simulink model "test_old_est"  (Simulink 6.2)
settings: Solver=ode45  StartTime=0.0  StopTime=10.0  RelTol=1e-3
libraries: xbsIndex_r3 x10, fft_library x1
settings Model: LastModifiedBy=mdexter
settings DebuggingCC: SolverPrmCheckMsg=warning

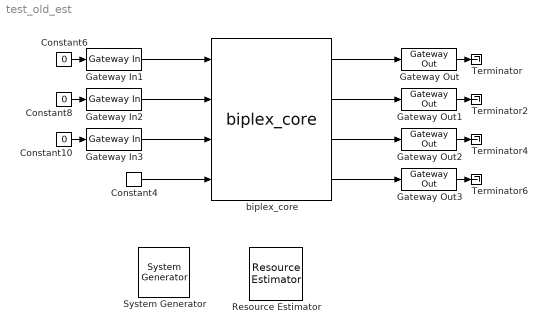
== system test_old_est ==
  " System Generator" : xbsIndex_r3/ System Generator  Tag=genX  xilinxfamily=Virtex2P  part=xc2vp40  speed=-6  package=ff1152  synthesis_tool=XST  directory=./test_old_est.netlist  testbench=off  simulink_period=1  sysclk_period=10  incr_netlist=off  trim_vbits=Everywhere in SubSystem  dbl_ovrd=According to Block Masks  core_generation=According to Block Masks  run_coregen=off  deprecated_control=off  eval_field=0
      settings: AttributesFormatString=System\nGenerator
  Constant10 : Constant  Value=0
  Constant4 : xbsIndex_r3/Constant  const=0  equ=P=C  arith_type=Unsigned  n_bits=10  bin_pt=0  opselect=C  inp2=PCIN>>17  opr=+  inp1=P  carry=CIN  iostate=0  explicit_period=on  period=1  dbl_ovrd=off
  Constant6 : Constant  Value=0
  Constant8 : Constant  Value=0
  Gateway In1 : xbsIndex_r3/Gateway In  arith_type=Unsigned  n_bits=36  bin_pt=0  quantization=Truncate  overflow=Wrap  period=1  timing_constraint=None  locs_specified=off  LOCs={}  needs_fixed_name=off  dbl_ovrd=off  show_param=off
      settings: xl_area=[0 0 0 0 36 0 0]
  Gateway In2 : xbsIndex_r3/Gateway In  arith_type=Unsigned  n_bits=36  bin_pt=0  quantization=Truncate  overflow=Wrap  period=1  timing_constraint=None  locs_specified=off  LOCs={}  needs_fixed_name=off  dbl_ovrd=off  show_param=off
      settings: xl_area=[0 0 0 0 36 0 0]
  Gateway In3 : xbsIndex_r3/Gateway In  arith_type=Boolean  n_bits=8  bin_pt=7  quantization=Truncate  overflow=Wrap  period=1  timing_constraint=None  locs_specified=off  LOCs={}  needs_fixed_name=off  dbl_ovrd=off  show_param=off
      settings: xl_area=[0 0 0 0 1 0 0]
  Gateway Out{,1..3} (4 alike) : xbsIndex_r3/Gateway Out  output_type=Double  nbits=8  bin_pt=6  arith_type=Boolean  quantization=Truncate  overflow=Wrap  hdl_port=on  timing_constraint=None  locs_specified=off  LOCs={}  needs_fixed_name=off  show_param=off
      Gateway Out settings: xl_area=[0 0 0 0 36 0 0]
      Gateway Out1 settings: xl_area=[0 0 0 0 36 0 0]
      Gateway Out2 settings: xl_area=[0 0 0 0 1 0 0]
      Gateway Out3 settings: xl_area=[0 0 0 0 1 0 0]
  Resource Estimator : xbsIndex_r3/Resource Estimator  Tag=resEstTag  xl_estimator_area=[5709 8870 8 9342 147 24 0]  xl_use_estimator_area=off  simulink_period=1  mrp_directory=./test_old_est.netlist
      settings: AttributesFormatString=Resource Estimator\n%<xl_estimator_area>\n[SL FF BR LUT IO MUL TBUF]
  Terminator{,2,4,6} (4 alike) : Terminator
  biplex_core : fft_library/biplex_core  FFTSize=10  BitWidth=18  quantization="Round  (unbiased: +/- Inf)"  overflow=Saturate  add_latency=1  mult_latency=3  bram_latency=1
      link override fft_stage_1/butterfly/Convert: quantization="Round  (unbiased: +/- Inf)"  overflow=Saturate
      link override fft_stage_1/butterfly/Convert1: quantization="Round  (unbiased: +/- Inf)"  overflow=Saturate
      link override fft_stage_1/butterfly/Convert2: quantization="Round  (unbiased: +/- Inf)"  overflow=Saturate
      link override fft_stage_1/butterfly/Convert3: quantization="Round  (unbiased: +/- Inf)"  overflow=Saturate
      link override fft_stage_1/delay_b/delay_bram/Constant2: equ=P=C
      link override fft_stage_1/delay_b/delay_im/delay_bram/Constant2: equ=P=C
      link override fft_stage_1/delay_b/delay_re/delay_bram/Constant2: equ=P=C
      link override fft_stage_1/delay_f/delay_bram/Constant2: equ=P=C
      link override fft_stage_1/delay_f/delay_im/delay_bram/Constant2: equ=P=C
      link override fft_stage_1/delay_f/delay_re/delay_bram/Constant2: equ=P=C
      link override fft_stage_1/sync_delay_x/Constant: equ=P=C
      link override fft_stage_1/sync_delay_x/Constant1: equ=P=C
      link override fft_stage_1/sync_delay_x/Constant2: equ=P=C
      link override fft_stage_1/sync_delay_x/Constant3: equ=P=C
      link override fft_stage_10/butterfly/Convert: quantization="Round  (unbiased: +/- Inf)"  overflow=Saturate
      link override fft_stage_10/butterfly/Convert1: quantization="Round  (unbiased: +/- Inf)"  overflow=Saturate
      link override fft_stage_10/butterfly/Convert2: quantization="Round  (unbiased: +/- Inf)"  overflow=Saturate
      link override fft_stage_10/butterfly/Convert3: quantization="Round  (unbiased: +/- Inf)"  overflow=Saturate
      link override fft_stage_10/butterfly/twiddle_general/br_coeff_gen/ROM: distributed_mem=off
      link override fft_stage_10/butterfly/twiddle_general/br_coeff_gen/ROM1: distributed_mem=off
      link override fft_stage_10/butterfly/twiddle_general_3mult/br_coeff_gen/ROM: distributed_mem=off
      link override fft_stage_10/butterfly/twiddle_general_3mult/br_coeff_gen/ROM1: distributed_mem=off
      link override fft_stage_10/sync_delay_x/Constant: equ=P=C
      link override fft_stage_10/sync_delay_x/Constant1: equ=P=C
      link override fft_stage_10/sync_delay_x/Constant2: equ=P=C
      link override fft_stage_10/sync_delay_x/Constant3: equ=P=C
      link override fft_stage_2/butterfly/Convert: quantization="Round  (unbiased: +/- Inf)"  overflow=Saturate
      link override fft_stage_2/butterfly/Convert1: quantization="Round  (unbiased: +/- Inf)"  overflow=Saturate
      link override fft_stage_2/butterfly/Convert2: quantization="Round  (unbiased: +/- Inf)"  overflow=Saturate
      link override fft_stage_2/butterfly/Convert3: quantization="Round  (unbiased: +/- Inf)"  overflow=Saturate
      link override fft_stage_2/delay_b/delay_bram/Constant2: equ=P=C
      link override fft_stage_2/delay_b/delay_im/delay_bram/Constant2: equ=P=C
      link override fft_stage_2/delay_b/delay_re/delay_bram/Constant2: equ=P=C
      link override fft_stage_2/delay_f/delay_bram/Constant2: equ=P=C
      link override fft_stage_2/delay_f/delay_im/delay_bram/Constant2: equ=P=C
      link override fft_stage_2/delay_f/delay_re/delay_bram/Constant2: equ=P=C
      link override fft_stage_2/sync_delay_x/Constant: equ=P=C
      link override fft_stage_2/sync_delay_x/Constant1: equ=P=C
      link override fft_stage_2/sync_delay_x/Constant2: equ=P=C
      link override fft_stage_2/sync_delay_x/Constant3: equ=P=C
      link override fft_stage_3/butterfly/Convert: quantization="Round  (unbiased: +/- Inf)"  overflow=Saturate
      link override fft_stage_3/butterfly/Convert1: quantization="Round  (unbiased: +/- Inf)"  overflow=Saturate
      link override fft_stage_3/butterfly/Convert2: quantization="Round  (unbiased: +/- Inf)"  overflow=Saturate
      link override fft_stage_3/butterfly/Convert3: quantization="Round  (unbiased: +/- Inf)"  overflow=Saturate
      link override fft_stage_3/delay_b/delay_im/delay_bram/Constant2: equ=P=C
      link override fft_stage_3/delay_b/delay_re/delay_bram/Constant2: equ=P=C
      link override fft_stage_3/delay_f/delay_im/delay_bram/Constant2: equ=P=C
      link override fft_stage_3/delay_f/delay_re/delay_bram/Constant2: equ=P=C
      link override fft_stage_3/sync_delay_x/Constant: equ=P=C
      link override fft_stage_3/sync_delay_x/Constant1: equ=P=C
      link override fft_stage_3/sync_delay_x/Constant2: equ=P=C
      link override fft_stage_3/sync_delay_x/Constant3: equ=P=C
      link override fft_stage_4/butterfly/Convert: quantization="Round  (unbiased: +/- Inf)"  overflow=Saturate
      link override fft_stage_4/butterfly/Convert1: quantization="Round  (unbiased: +/- Inf)"  overflow=Saturate
      link override fft_stage_4/butterfly/Convert2: quantization="Round  (unbiased: +/- Inf)"  overflow=Saturate
      link override fft_stage_4/butterfly/Convert3: quantization="Round  (unbiased: +/- Inf)"  overflow=Saturate
      link override fft_stage_4/delay_b/delay_im/delay_bram/Constant2: equ=P=C
      link override fft_stage_4/delay_b/delay_re/delay_bram/Constant2: equ=P=C
      link override fft_stage_4/delay_f/delay_im/delay_bram/Constant2: equ=P=C
      link override fft_stage_4/delay_f/delay_re/delay_bram/Constant2: equ=P=C
      link override fft_stage_4/sync_delay_x/Constant: equ=P=C
      link override fft_stage_4/sync_delay_x/Constant1: equ=P=C
      link override fft_stage_4/sync_delay_x/Constant2: equ=P=C
      link override fft_stage_4/sync_delay_x/Constant3: equ=P=C
      link override fft_stage_5/butterfly/Convert: quantization="Round  (unbiased: +/- Inf)"  overflow=Saturate
      link override fft_stage_5/butterfly/Convert1: quantization="Round  (unbiased: +/- Inf)"  overflow=Saturate
      link override fft_stage_5/butterfly/Convert2: quantization="Round  (unbiased: +/- Inf)"  overflow=Saturate
      link override fft_stage_5/butterfly/Convert3: quantization="Round  (unbiased: +/- Inf)"  overflow=Saturate
      link override fft_stage_5/sync_delay_x/Constant: equ=P=C
      link override fft_stage_5/sync_delay_x/Constant1: equ=P=C
      link override fft_stage_5/sync_delay_x/Constant2: equ=P=C
      link override fft_stage_5/sync_delay_x/Constant3: equ=P=C
      link override fft_stage_6/butterfly/Convert: quantization="Round  (unbiased: +/- Inf)"  overflow=Saturate
      link override fft_stage_6/butterfly/Convert1: quantization="Round  (unbiased: +/- Inf)"  overflow=Saturate
      link override fft_stage_6/butterfly/Convert2: quantization="Round  (unbiased: +/- Inf)"  overflow=Saturate
      link override fft_stage_6/butterfly/Convert3: quantization="Round  (unbiased: +/- Inf)"  overflow=Saturate
      link override fft_stage_6/sync_delay_x/Constant: equ=P=C
      link override fft_stage_6/sync_delay_x/Constant1: equ=P=C
      link override fft_stage_6/sync_delay_x/Constant2: equ=P=C
      link override fft_stage_6/sync_delay_x/Constant3: equ=P=C
      link override fft_stage_7/butterfly/Convert: quantization="Round  (unbiased: +/- Inf)"  overflow=Saturate
      link override fft_stage_7/butterfly/Convert1: quantization="Round  (unbiased: +/- Inf)"  overflow=Saturate
      link override fft_stage_7/butterfly/Convert2: quantization="Round  (unbiased: +/- Inf)"  overflow=Saturate
      link override fft_stage_7/butterfly/Convert3: quantization="Round  (unbiased: +/- Inf)"  overflow=Saturate
      link override fft_stage_7/sync_delay_x/Constant: equ=P=C
      link override fft_stage_7/sync_delay_x/Constant1: equ=P=C
      link override fft_stage_7/sync_delay_x/Constant2: equ=P=C
      link override fft_stage_7/sync_delay_x/Constant3: equ=P=C
      link override fft_stage_8/butterfly/Convert: quantization="Round  (unbiased: +/- Inf)"  overflow=Saturate
      link override fft_stage_8/butterfly/Convert1: quantization="Round  (unbiased: +/- Inf)"  overflow=Saturate
      link override fft_stage_8/butterfly/Convert2: quantization="Round  (unbiased: +/- Inf)"  overflow=Saturate
      link override fft_stage_8/butterfly/Convert3: quantization="Round  (unbiased: +/- Inf)"  overflow=Saturate
      link override fft_stage_8/sync_delay_x/Constant: equ=P=C
      link override fft_stage_8/sync_delay_x/Constant1: equ=P=C
      link override fft_stage_8/sync_delay_x/Constant2: equ=P=C
      link override fft_stage_8/sync_delay_x/Constant3: equ=P=C
      link override fft_stage_9/butterfly/Convert: quantization="Round  (unbiased: +/- Inf)"  overflow=Saturate
      link override fft_stage_9/butterfly/Convert1: quantization="Round  (unbiased: +/- Inf)"  overflow=Saturate
      link override fft_stage_9/butterfly/Convert2: quantization="Round  (unbiased: +/- Inf)"  overflow=Saturate
      link override fft_stage_9/butterfly/Convert3: quantization="Round  (unbiased: +/- Inf)"  overflow=Saturate
      link override fft_stage_9/butterfly/twiddle_general/br_coeff_gen/ROM: distributed_mem=off
      link override fft_stage_9/butterfly/twiddle_general/br_coeff_gen/ROM1: distributed_mem=off
      link override fft_stage_9/butterfly/twiddle_general_3mult/br_coeff_gen/ROM: distributed_mem=off
      link override fft_stage_9/butterfly/twiddle_general_3mult/br_coeff_gen/ROM1: distributed_mem=off
      link override fft_stage_9/sync_delay_x/Constant: equ=P=C
      link override fft_stage_9/sync_delay_x/Constant1: equ=P=C
      link override fft_stage_9/sync_delay_x/Constant2: equ=P=C
      link override fft_stage_9/sync_delay_x/Constant3: equ=P=C
      link override fft_stage_1/Counter: xl_area=[5 10 0 10 0 0 0]
      link override fft_stage_1/Delay: xl_area=[1 1 0 0 0 0 0]
      link override fft_stage_1/Mux: xl_area=[18 36 0 36 0 0 0]
      link override fft_stage_1/Mux1: xl_area=[18 36 0 36 0 0 0]
      link override fft_stage_1/butterfly/AddSub: xl_area=[10 19 0 19 0 0 0]
      link override fft_stage_1/butterfly/AddSub1: xl_area=[10 19 0 19 0 0 0]
      link override fft_stage_1/butterfly/AddSub2: xl_area=[10 19 0 19 0 0 0]
      link override fft_stage_1/butterfly/AddSub3: xl_area=[10 19 0 19 0 0 0]
      link override fft_stage_1/butterfly/Convert: xl_area=[29 18 0 57 0 0 0]
      link override fft_stage_1/butterfly/Convert1: xl_area=[29 18 0 57 0 0 0]
      link override fft_stage_1/butterfly/Convert2: xl_area=[29 18 0 57 0 0 0]
      link override fft_stage_1/butterfly/Convert3: xl_area=[29 18 0 57 0 0 0]
      link override fft_stage_1/butterfly/Delay: xl_area=[1 1 0 1 0 0 0]
      link override fft_stage_1/butterfly/Delay3: xl_area=[1 1 0 0 0 0 0]
      link override fft_stage_1/butterfly/Inverter: xl_area=[0 0 0 0 0 0 0]
      link override fft_stage_1/butterfly/Logical: xl_area=[1 1 0 1 0 0 0]
      link override fft_stage_1/butterfly/Logical1: xl_area=[1 1 0 1 0 0 0]
      link override fft_stage_1/butterfly/Logical10: xl_area=[1 1 0 1 0 0 0]
      link override fft_stage_1/butterfly/Logical11: xl_area=[1 1 0 1 0 0 0]
      link override fft_stage_1/butterfly/Logical12: xl_area=[1 1 0 1 0 0 0]
      link override fft_stage_1/butterfly/Logical13: xl_area=[1 1 0 1 0 0 0]
      link override fft_stage_1/butterfly/Logical2: xl_area=[1 1 0 1 0 0 0]
      link override fft_stage_1/butterfly/Logical3: xl_area=[1 1 0 1 0 0 0]
      link override fft_stage_1/butterfly/Logical4: xl_area=[1 1 0 1 0 0 0]
      link override fft_stage_1/butterfly/Logical5: xl_area=[1 1 0 1 0 0 0]
      link override fft_stage_1/butterfly/Logical6: xl_area=[1 1 0 1 0 0 0]
      link override fft_stage_1/butterfly/Logical7: xl_area=[1 1 0 1 0 0 0]
      link override fft_stage_1/butterfly/Logical8: xl_area=[1 1 0 1 0 0 0]
      link override fft_stage_1/butterfly/Logical9: xl_area=[1 1 0 1 0 0 0]
      link override fft_stage_1/butterfly/Mux: xl_area=[10 20 0 20 0 0 0]
      link override fft_stage_1/butterfly/Mux1: xl_area=[10 20 0 20 0 0 0]
      link override fft_stage_1/butterfly/Mux2: xl_area=[10 20 0 20 0 0 0]
      link override fft_stage_1/butterfly/Mux3: xl_area=[10 20 0 20 0 0 0]
      link override fft_stage_1/delay_b/delay_bram/Counter: xl_area=[7 9 0 12 0 0 0]
      link override fft_stage_1/delay_b/delay_bram/Single Port RAM: xl_area=[0 0 1 0 0 0 0]
      link override fft_stage_1/delay_b/delay_im/delay_bram/Counter: xl_area=[7 9 0 12 0 0 0]
      link override fft_stage_1/delay_b/delay_im/delay_bram/Single Port RAM: xl_area=[0 0 1 0 0 0 0]
      link override fft_stage_1/delay_b/delay_re/delay_bram/Counter: xl_area=[7 9 0 12 0 0 0]
      link override fft_stage_1/delay_b/delay_re/delay_bram/Single Port RAM: xl_area=[0 0 1 0 0 0 0]
      link override fft_stage_1/delay_f/delay_bram/Counter: xl_area=[7 9 0 12 0 0 0]
      link override fft_stage_1/delay_f/delay_bram/Single Port RAM: xl_area=[0 0 1 0 0 0 0]
      link override fft_stage_1/delay_f/delay_im/delay_bram/Counter: xl_area=[7 9 0 12 0 0 0]
      link override fft_stage_1/delay_f/delay_im/delay_bram/Single Port RAM: xl_area=[0 0 1 0 0 0 0]
      link override fft_stage_1/delay_f/delay_re/delay_bram/Counter: xl_area=[7 9 0 12 0 0 0]
      link override fft_stage_1/delay_f/delay_re/delay_bram/Single Port RAM: xl_area=[0 0 1 0 0 0 0]
      link override fft_stage_1/sync_delay_x/Counter: xl_area=[6 10 0 11 0 0 0]
      link override fft_stage_1/sync_delay_x/Logical: xl_area=[1 0 0 1 0 0 0]
      link override fft_stage_1/sync_delay_x/Mux: xl_area=[1 0 0 1 0 0 0]
      link override fft_stage_1/sync_delay_x/Relational: xl_area=[3 0 0 5 0 0 0]
      link override fft_stage_1/sync_delay_x/Relational1: xl_area=[3 0 0 5 0 0 0]
      link override fft_stage_10/Counter: xl_area=[2 1 0 1 0 0 0]
      link override fft_stage_10/Delay: xl_area=[1 1 0 0 0 0 0]
      link override fft_stage_10/Logical1: xl_area=[1 1 0 1 0 0 0]
      link override fft_stage_10/Mux: xl_area=[18 36 0 36 0 0 0]
      link override fft_stage_10/Mux1: xl_area=[18 36 0 36 0 0 0]
      link override fft_stage_10/butterfly/AddSub: xl_area=[12 23 0 23 0 0 0]
      link override fft_stage_10/butterfly/AddSub1: xl_area=[12 23 0 23 0 0 0]
      link override fft_stage_10/butterfly/AddSub2: xl_area=[12 23 0 23 0 0 0]
      link override fft_stage_10/butterfly/AddSub3: xl_area=[12 23 0 23 0 0 0]
      link override fft_stage_10/butterfly/Convert: xl_area=[31 18 0 61 0 0 0]
      link override fft_stage_10/butterfly/Convert1: xl_area=[31 18 0 61 0 0 0]
      link override fft_stage_10/butterfly/Convert2: xl_area=[31 18 0 61 0 0 0]
      link override fft_stage_10/butterfly/Convert3: xl_area=[31 18 0 61 0 0 0]
      link override fft_stage_10/butterfly/Delay: xl_area=[1 1 0 1 0 0 0]
      link override fft_stage_10/butterfly/Delay3: xl_area=[1 1 0 0 0 0 0]
      link override fft_stage_10/butterfly/Inverter: xl_area=[0 0 0 0 0 0 0]
      link override fft_stage_10/butterfly/Logical: xl_area=[1 1 0 1 0 0 0]
      link override fft_stage_10/butterfly/Logical1: xl_area=[1 1 0 1 0 0 0]
      link override fft_stage_10/butterfly/Logical10: xl_area=[1 1 0 1 0 0 0]
      link override fft_stage_10/butterfly/Logical11: xl_area=[1 1 0 1 0 0 0]
      link override fft_stage_10/butterfly/Logical12: xl_area=[1 1 0 1 0 0 0]
      link override fft_stage_10/butterfly/Logical13: xl_area=[1 1 0 1 0 0 0]
      link override fft_stage_10/butterfly/Logical2: xl_area=[1 1 0 1 0 0 0]
      link override fft_stage_10/butterfly/Logical3: xl_area=[1 1 0 1 0 0 0]
      link override fft_stage_10/butterfly/Logical4: xl_area=[1 1 0 1 0 0 0]
      link override fft_stage_10/butterfly/Logical5: xl_area=[1 1 0 1 0 0 0]
      link override fft_stage_10/butterfly/Logical6: xl_area=[1 1 0 1 0 0 0]
      link override fft_stage_10/butterfly/Logical7: xl_area=[1 1 0 1 0 0 0]
      link override fft_stage_10/butterfly/Logical8: xl_area=[1 1 0 1 0 0 0]
      link override fft_stage_10/butterfly/Logical9: xl_area=[1 1 0 1 0 0 0]
      link override fft_stage_10/butterfly/Mux: xl_area=[12 24 0 24 0 0 0]
      link override fft_stage_10/butterfly/Mux1: xl_area=[12 24 0 24 0 0 0]
      link override fft_stage_10/butterfly/Mux2: xl_area=[12 24 0 24 0 0 0]
      link override fft_stage_10/butterfly/Mux3: xl_area=[12 24 0 24 0 0 0]
      link override fft_stage_10/butterfly/twiddle_general/AddSub: xl_area=[11 21 0 21 0 0 0]
      link override fft_stage_10/butterfly/twiddle_general/AddSub1: xl_area=[11 21 0 21 0 0 0]
      link override fft_stage_10/butterfly/twiddle_general/Convert: xl_area=[0 0 0 0 0 0 0]
      link override fft_stage_10/butterfly/twiddle_general/Convert1: xl_area=[0 0 0 0 0 0 0]
      link override fft_stage_10/butterfly/twiddle_general/Convert2: xl_area=[0 0 0 0 0 0 0]
      link override fft_stage_10/butterfly/twiddle_general/Convert3: xl_area=[0 0 0 0 0 0 0]
      link override fft_stage_10/butterfly/twiddle_general/Delay: xl_area=[18 36 0 36 0 0 0]
      link override fft_stage_10/butterfly/twiddle_general/Delay1: xl_area=[18 36 0 0 0 0 0]
      link override fft_stage_10/butterfly/twiddle_general/Delay2: xl_area=[1 1 0 1 0 0 0]
      link override fft_stage_10/butterfly/twiddle_general/Mult: xl_area=[36 72 0 36 0 1 0]
      link override fft_stage_10/butterfly/twiddle_general/Mult1: xl_area=[36 72 0 36 0 1 0]
      link override fft_stage_10/butterfly/twiddle_general/Mult2: xl_area=[36 72 0 36 0 1 0]
      link override fft_stage_10/butterfly/twiddle_general/Mult3: xl_area=[36 72 0 36 0 1 0]
      link override fft_stage_10/butterfly/twiddle_general/br_coeff_gen/Counter: xl_area=[5 9 0 9 0 0 0]
      link override fft_stage_10/butterfly/twiddle_general/br_coeff_gen/ROM: xl_area=[0 0 1 0 0 0 0]
      link override fft_stage_10/butterfly/twiddle_general/br_coeff_gen/ROM1: xl_area=[0 0 1 0 0 0 0]
      link override fft_stage_10/butterfly/twiddle_general_3mult/AddSub: xl_area=[11 22 0 22 0 0 0]
      link override fft_stage_10/butterfly/twiddle_general_3mult/AddSub1: xl_area=[10 19 0 19 0 0 0]
      link override fft_stage_10/butterfly/twiddle_general_3mult/AddSub2: xl_area=[10 19 0 19 0 0 0]
      link override fft_stage_10/butterfly/twiddle_general_3mult/AddSub3: xl_area=[10 19 0 19 0 0 0]
      link override fft_stage_10/butterfly/twiddle_general_3mult/AddSub4: xl_area=[11 22 0 22 0 0 0]
      link override fft_stage_10/butterfly/twiddle_general_3mult/Convert: xl_area=[0 0 0 0 0 0 0]
      link override fft_stage_10/butterfly/twiddle_general_3mult/Convert1: xl_area=[0 0 0 0 0 0 0]
      link override fft_stage_10/butterfly/twiddle_general_3mult/Convert2: xl_area=[0 0 0 0 0 0 0]
      link override fft_stage_10/butterfly/twiddle_general_3mult/Convert3: xl_area=[0 0 0 0 0 0 0]
      link override fft_stage_10/butterfly/twiddle_general_3mult/Convert4: xl_area=[0 0 0 0 0 0 0]
      link override fft_stage_10/butterfly/twiddle_general_3mult/Convert5: xl_area=[0 0 0 0 0 0 0]
      link override fft_stage_10/butterfly/twiddle_general_3mult/Delay: xl_area=[18 36 0 36 0 0 0]
      link override fft_stage_10/butterfly/twiddle_general_3mult/Delay1: xl_area=[18 36 0 0 0 0 0]
      link override fft_stage_10/butterfly/twiddle_general_3mult/Delay2: xl_area=[1 1 0 1 0 0 0]
      link override fft_stage_10/butterfly/twiddle_general_3mult/Delay3: xl_area=[9 18 0 0 0 0 0]
      link override fft_stage_10/butterfly/twiddle_general_3mult/Delay4: xl_area=[9 18 0 0 0 0 0]
      link override fft_stage_10/butterfly/twiddle_general_3mult/Delay5: xl_area=[9 18 0 0 0 0 0]
      link override fft_stage_10/butterfly/twiddle_general_3mult/Mult: xl_area=[36 72 0 36 0 1 0]
      link override fft_stage_10/butterfly/twiddle_general_3mult/Mult1: xl_area=[36 72 0 36 0 1 0]
      link override fft_stage_10/butterfly/twiddle_general_3mult/Mult2: xl_area=[36 72 0 36 0 1 0]
      link override fft_stage_10/butterfly/twiddle_general_3mult/br_coeff_gen/Counter: xl_area=[5 9 0 9 0 0 0]
      link override fft_stage_10/butterfly/twiddle_general_3mult/br_coeff_gen/ROM: xl_area=[0 0 1 0 0 0 0]
      link override fft_stage_10/butterfly/twiddle_general_3mult/br_coeff_gen/ROM1: xl_area=[0 0 1 0 0 0 0]
      link override fft_stage_10/delay_b/delay_im/delay_slr/delay_slr: xl_area=[9 18 0 0 0 0 0]
      link override fft_stage_10/delay_b/delay_re/delay_slr/delay_slr: xl_area=[9 18 0 0 0 0 0]
      link override fft_stage_10/delay_b/delay_slr/delay_slr: xl_area=[18 36 0 0 0 0 0]
      link override fft_stage_10/delay_f/delay_im/delay_slr/delay_slr: xl_area=[9 18 0 0 0 0 0]
      link override fft_stage_10/delay_f/delay_re/delay_slr/delay_slr: xl_area=[9 18 0 0 0 0 0]
      link override fft_stage_10/delay_f/delay_slr/delay_slr: xl_area=[18 36 0 0 0 0 0]
      link override fft_stage_10/sync_delay_x/Counter: xl_area=[2 2 0 3 0 0 0]
      link override fft_stage_10/sync_delay_x/Logical: xl_area=[1 0 0 1 0 0 0]
      link override fft_stage_10/sync_delay_x/Mux: xl_area=[1 0 0 1 0 0 0]
      link override fft_stage_10/sync_delay_x/Relational: xl_area=[1 0 0 1 0 0 0]
      link override fft_stage_10/sync_delay_x/Relational1: xl_area=[1 0 0 1 0 0 0]
      link override fft_stage_2/Counter: xl_area=[5 9 0 9 0 0 0]
      link override fft_stage_2/Delay: xl_area=[1 1 0 0 0 0 0]
      link override fft_stage_2/Logical1: xl_area=[1 1 0 1 0 0 0]
      link override fft_stage_2/Mux: xl_area=[18 36 0 36 0 0 0]
      link override fft_stage_2/Mux1: xl_area=[18 36 0 36 0 0 0]
      link override fft_stage_2/butterfly/AddSub: xl_area=[10 19 0 19 0 0 0]
      link override fft_stage_2/butterfly/AddSub1: xl_area=[10 19 0 19 0 0 0]
      link override fft_stage_2/butterfly/AddSub2: xl_area=[10 19 0 19 0 0 0]
      link override fft_stage_2/butterfly/AddSub3: xl_area=[10 19 0 19 0 0 0]
      link override fft_stage_2/butterfly/Convert: xl_area=[29 18 0 57 0 0 0]
      link override fft_stage_2/butterfly/Convert1: xl_area=[29 18 0 57 0 0 0]
      link override fft_stage_2/butterfly/Convert2: xl_area=[29 18 0 57 0 0 0]
      link override fft_stage_2/butterfly/Convert3: xl_area=[29 18 0 57 0 0 0]
      link override fft_stage_2/butterfly/Delay: xl_area=[1 1 0 1 0 0 0]
      link override fft_stage_2/butterfly/Delay3: xl_area=[1 1 0 0 0 0 0]
      link override fft_stage_2/butterfly/Inverter: xl_area=[0 0 0 0 0 0 0]
      link override fft_stage_2/butterfly/Logical: xl_area=[1 1 0 1 0 0 0]
      link override fft_stage_2/butterfly/Logical1: xl_area=[1 1 0 1 0 0 0]
      link override fft_stage_2/butterfly/Logical10: xl_area=[1 1 0 1 0 0 0]
      link override fft_stage_2/butterfly/Logical11: xl_area=[1 1 0 1 0 0 0]
      link override fft_stage_2/butterfly/Logical12: xl_area=[1 1 0 1 0 0 0]
      link override fft_stage_2/butterfly/Logical13: xl_area=[1 1 0 1 0 0 0]
      link override fft_stage_2/butterfly/Logical2: xl_area=[1 1 0 1 0 0 0]
      link override fft_stage_2/butterfly/Logical3: xl_area=[1 1 0 1 0 0 0]
      link override fft_stage_2/butterfly/Logical4: xl_area=[1 1 0 1 0 0 0]
      link override fft_stage_2/butterfly/Logical5: xl_area=[1 1 0 1 0 0 0]
      link override fft_stage_2/butterfly/Logical6: xl_area=[1 1 0 1 0 0 0]
      link override fft_stage_2/butterfly/Logical7: xl_area=[1 1 0 1 0 0 0]
      link override fft_stage_2/butterfly/Logical8: xl_area=[1 1 0 1 0 0 0]
      link override fft_stage_2/butterfly/Logical9: xl_area=[1 1 0 1 0 0 0]
      link override fft_stage_2/butterfly/Mux: xl_area=[10 20 0 20 0 0 0]
      link override fft_stage_2/butterfly/Mux1: xl_area=[10 20 0 20 0 0 0]
      link override fft_stage_2/butterfly/Mux2: xl_area=[10 20 0 20 0 0 0]
      link override fft_stage_2/butterfly/Mux3: xl_area=[10 20 0 20 0 0 0]
      link override fft_stage_2/butterfly/twiddle_stage_2/Counter: xl_area=[5 9 0 9 0 0 0]
      link override fft_stage_2/butterfly/twiddle_stage_2/Delay: xl_area=[18 36 0 0 0 0 0]
      link override fft_stage_2/butterfly/twiddle_stage_2/Delay2: xl_area=[1 1 0 0 0 0 0]
      link override fft_stage_2/butterfly/twiddle_stage_2/Mux: xl_area=[9 18 0 18 0 0 0]
      link override fft_stage_2/butterfly/twiddle_stage_2/Mux1: xl_area=[9 18 0 18 0 0 0]
      link override fft_stage_2/butterfly/twiddle_stage_2/Negate1: xl_area=[9 0 0 18 0 0 0]
      link override fft_stage_2/delay_b/delay_bram/Counter: xl_area=[6 8 0 11 0 0 0]
      link override fft_stage_2/delay_b/delay_bram/Single Port RAM: xl_area=[0 0 1 0 0 0 0]
      link override fft_stage_2/delay_b/delay_im/delay_bram/Counter: xl_area=[6 8 0 11 0 0 0]
      link override fft_stage_2/delay_b/delay_im/delay_bram/Single Port RAM: xl_area=[0 0 1 0 0 0 0]
      link override fft_stage_2/delay_b/delay_re/delay_bram/Counter: xl_area=[6 8 0 11 0 0 0]
      link override fft_stage_2/delay_b/delay_re/delay_bram/Single Port RAM: xl_area=[0 0 1 0 0 0 0]
      link override fft_stage_2/delay_f/delay_bram/Counter: xl_area=[6 8 0 11 0 0 0]
      link override fft_stage_2/delay_f/delay_bram/Single Port RAM: xl_area=[0 0 1 0 0 0 0]
      link override fft_stage_2/delay_f/delay_im/delay_bram/Counter: xl_area=[6 8 0 11 0 0 0]
      link override fft_stage_2/delay_f/delay_im/delay_bram/Single Port RAM: xl_area=[0 0 1 0 0 0 0]
      link override fft_stage_2/delay_f/delay_re/delay_bram/Counter: xl_area=[6 8 0 11 0 0 0]
      link override fft_stage_2/delay_f/delay_re/delay_bram/Single Port RAM: xl_area=[0 0 1 0 0 0 0]
      link override fft_stage_2/sync_delay_x/Counter: xl_area=[5 9 0 10 0 0 0]
      link override fft_stage_2/sync_delay_x/Logical: xl_area=[1 0 0 1 0 0 0]
      link override fft_stage_2/sync_delay_x/Mux: xl_area=[1 0 0 1 0 0 0]
      link override fft_stage_2/sync_delay_x/Relational: xl_area=[3 0 0 5 0 0 0]
      link override fft_stage_2/sync_delay_x/Relational1: xl_area=[3 0 0 5 0 0 0]
      link override fft_stage_3/Counter: xl_area=[4 8 0 8 0 0 0]
      link override fft_stage_3/Delay: xl_area=[1 1 0 0 0 0 0]
      link override fft_stage_3/Logical1: xl_area=[1 1 0 1 0 0 0]
      link override fft_stage_3/Mux: xl_area=[18 36 0 36 0 0 0]
      link override fft_stage_3/Mux1: xl_area=[18 36 0 36 0 0 0]
      link override fft_stage_3/butterfly/AddSub: xl_area=[12 23 0 23 0 0 0]
      link override fft_stage_3/butterfly/AddSub1: xl_area=[12 23 0 23 0 0 0]
      link override fft_stage_3/butterfly/AddSub2: xl_area=[12 23 0 23 0 0 0]
      link override fft_stage_3/butterfly/AddSub3: xl_area=[12 23 0 23 0 0 0]
      link override fft_stage_3/butterfly/Convert: xl_area=[31 18 0 61 0 0 0]
      link override fft_stage_3/butterfly/Convert1: xl_area=[31 18 0 61 0 0 0]
      link override fft_stage_3/butterfly/Convert2: xl_area=[31 18 0 61 0 0 0]
      link override fft_stage_3/butterfly/Convert3: xl_area=[31 18 0 61 0 0 0]
      link override fft_stage_3/butterfly/Delay: xl_area=[1 1 0 1 0 0 0]
      link override fft_stage_3/butterfly/Delay3: xl_area=[1 1 0 0 0 0 0]
      link override fft_stage_3/butterfly/Inverter: xl_area=[0 0 0 0 0 0 0]
      link override fft_stage_3/butterfly/Logical: xl_area=[1 1 0 1 0 0 0]
      link override fft_stage_3/butterfly/Logical1: xl_area=[1 1 0 1 0 0 0]
      link override fft_stage_3/butterfly/Logical10: xl_area=[1 1 0 1 0 0 0]
      link override fft_stage_3/butterfly/Logical11: xl_area=[1 1 0 1 0 0 0]
      link override fft_stage_3/butterfly/Logical12: xl_area=[1 1 0 1 0 0 0]
      link override fft_stage_3/butterfly/Logical13: xl_area=[1 1 0 1 0 0 0]
      link override fft_stage_3/butterfly/Logical2: xl_area=[1 1 0 1 0 0 0]
      link override fft_stage_3/butterfly/Logical3: xl_area=[1 1 0 1 0 0 0]
      link override fft_stage_3/butterfly/Logical4: xl_area=[1 1 0 1 0 0 0]
      link override fft_stage_3/butterfly/Logical5: xl_area=[1 1 0 1 0 0 0]
      link override fft_stage_3/butterfly/Logical6: xl_area=[1 1 0 1 0 0 0]
      link override fft_stage_3/butterfly/Logical7: xl_area=[1 1 0 1 0 0 0]
      link override fft_stage_3/butterfly/Logical8: xl_area=[1 1 0 1 0 0 0]
      link override fft_stage_3/butterfly/Logical9: xl_area=[1 1 0 1 0 0 0]
      link override fft_stage_3/butterfly/Mux: xl_area=[12 24 0 24 0 0 0]
      link override fft_stage_3/butterfly/Mux1: xl_area=[12 24 0 24 0 0 0]
      link override fft_stage_3/butterfly/Mux2: xl_area=[12 24 0 24 0 0 0]
      link override fft_stage_3/butterfly/Mux3: xl_area=[12 24 0 24 0 0 0]
      link override fft_stage_3/butterfly/twiddle_general/AddSub: xl_area=[11 21 0 21 0 0 0]
      link override fft_stage_3/butterfly/twiddle_general/AddSub1: xl_area=[11 21 0 21 0 0 0]
      link override fft_stage_3/butterfly/twiddle_general/Convert: xl_area=[0 0 0 0 0 0 0]
      link override fft_stage_3/butterfly/twiddle_general/Convert1: xl_area=[0 0 0 0 0 0 0]
      link override fft_stage_3/butterfly/twiddle_general/Convert2: xl_area=[0 0 0 0 0 0 0]
      link override fft_stage_3/butterfly/twiddle_general/Convert3: xl_area=[0 0 0 0 0 0 0]
      link override fft_stage_3/butterfly/twiddle_general/Delay: xl_area=[18 36 0 36 0 0 0]
      link override fft_stage_3/butterfly/twiddle_general/Delay1: xl_area=[18 36 0 0 0 0 0]
      link override fft_stage_3/butterfly/twiddle_general/Delay2: xl_area=[1 1 0 1 0 0 0]
      link override fft_stage_3/butterfly/twiddle_general/Mult: xl_area=[36 72 0 36 0 1 0]
      link override fft_stage_3/butterfly/twiddle_general/Mult1: xl_area=[36 72 0 36 0 1 0]
      link override fft_stage_3/butterfly/twiddle_general/Mult2: xl_area=[36 72 0 36 0 1 0]
      link override fft_stage_3/butterfly/twiddle_general/Mult3: xl_area=[36 72 0 36 0 1 0]
      link override fft_stage_3/butterfly/twiddle_general/br_coeff_gen/Counter: xl_area=[5 9 0 9 0 0 0]
      link override fft_stage_3/butterfly/twiddle_general/br_coeff_gen/ROM: xl_area=[9 18 0 18 0 0 0]
      link override fft_stage_3/butterfly/twiddle_general/br_coeff_gen/ROM1: xl_area=[9 18 0 11 0 0 0]
      link override fft_stage_3/butterfly/twiddle_general_3mult/AddSub: xl_area=[11 22 0 22 0 0 0]
      link override fft_stage_3/butterfly/twiddle_general_3mult/AddSub1: xl_area=[10 19 0 19 0 0 0]
      link override fft_stage_3/butterfly/twiddle_general_3mult/AddSub2: xl_area=[10 19 0 19 0 0 0]
      link override fft_stage_3/butterfly/twiddle_general_3mult/AddSub3: xl_area=[10 19 0 19 0 0 0]
      link override fft_stage_3/butterfly/twiddle_general_3mult/AddSub4: xl_area=[11 22 0 22 0 0 0]
      link override fft_stage_3/butterfly/twiddle_general_3mult/Convert: xl_area=[0 0 0 0 0 0 0]
      link override fft_stage_3/butterfly/twiddle_general_3mult/Convert1: xl_area=[0 0 0 0 0 0 0]
      link override fft_stage_3/butterfly/twiddle_general_3mult/Convert2: xl_area=[0 0 0 0 0 0 0]
      link override fft_stage_3/butterfly/twiddle_general_3mult/Convert3: xl_area=[0 0 0 0 0 0 0]
      link override fft_stage_3/butterfly/twiddle_general_3mult/Convert4: xl_area=[0 0 0 0 0 0 0]
      link override fft_stage_3/butterfly/twiddle_general_3mult/Convert5: xl_area=[0 0 0 0 0 0 0]
      link override fft_stage_3/butterfly/twiddle_general_3mult/Delay: xl_area=[18 36 0 36 0 0 0]
      link override fft_stage_3/butterfly/twiddle_general_3mult/Delay1: xl_area=[18 36 0 0 0 0 0]
      link override fft_stage_3/butterfly/twiddle_general_3mult/Delay2: xl_area=[1 1 0 1 0 0 0]
      link override fft_stage_3/butterfly/twiddle_general_3mult/Delay3: xl_area=[9 18 0 0 0 0 0]
      link override fft_stage_3/butterfly/twiddle_general_3mult/Delay4: xl_area=[9 18 0 0 0 0 0]
      link override fft_stage_3/butterfly/twiddle_general_3mult/Delay5: xl_area=[9 18 0 0 0 0 0]
      link override fft_stage_3/butterfly/twiddle_general_3mult/Mult: xl_area=[36 72 0 36 0 1 0]
      link override fft_stage_3/butterfly/twiddle_general_3mult/Mult1: xl_area=[36 72 0 36 0 1 0]
      link override fft_stage_3/butterfly/twiddle_general_3mult/Mult2: xl_area=[36 72 0 36 0 1 0]
      link override fft_stage_3/butterfly/twiddle_general_3mult/br_coeff_gen/Counter: xl_area=[5 9 0 9 0 0 0]
      link override fft_stage_3/butterfly/twiddle_general_3mult/br_coeff_gen/ROM: xl_area=[9 18 0 18 0 0 0]
      link override fft_stage_3/butterfly/twiddle_general_3mult/br_coeff_gen/ROM1: xl_area=[9 18 0 11 0 0 0]
      link override fft_stage_3/delay_b/delay_im/delay_bram/Counter: xl_area=[5 7 0 9 0 0 0]
      link override fft_stage_3/delay_b/delay_im/delay_bram/Single Port RAM: xl_area=[0 0 1 0 0 0 0]
      link override fft_stage_3/delay_b/delay_re/delay_bram/Counter: xl_area=[5 7 0 9 0 0 0]
      link override fft_stage_3/delay_b/delay_re/delay_bram/Single Port RAM: xl_area=[0 0 1 0 0 0 0]
      link override fft_stage_3/delay_b/delay_slr/delay_slr: xl_area=[144 288 0 288 0 0 0]
      link override fft_stage_3/delay_f/delay_im/delay_bram/Counter: xl_area=[5 7 0 9 0 0 0]
      link override fft_stage_3/delay_f/delay_im/delay_bram/Single Port RAM: xl_area=[0 0 1 0 0 0 0]
      link override fft_stage_3/delay_f/delay_re/delay_bram/Counter: xl_area=[5 7 0 9 0 0 0]
      link override fft_stage_3/delay_f/delay_re/delay_bram/Single Port RAM: xl_area=[0 0 1 0 0 0 0]
      link override fft_stage_3/delay_f/delay_slr/delay_slr: xl_area=[144 288 0 288 0 0 0]
      link override fft_stage_3/sync_delay_x/Counter: xl_area=[5 8 0 9 0 0 0]
      link override fft_stage_3/sync_delay_x/Logical: xl_area=[1 0 0 1 0 0 0]
      link override fft_stage_3/sync_delay_x/Mux: xl_area=[1 0 0 1 0 0 0]
      link override fft_stage_3/sync_delay_x/Relational: xl_area=[2 0 0 4 0 0 0]
      link override fft_stage_3/sync_delay_x/Relational1: xl_area=[2 0 0 4 0 0 0]
      link override fft_stage_4/Counter: xl_area=[4 7 0 7 0 0 0]
      link override fft_stage_4/Delay: xl_area=[1 1 0 0 0 0 0]
      link override fft_stage_4/Logical1: xl_area=[1 1 0 1 0 0 0]
      link override fft_stage_4/Mux: xl_area=[18 36 0 36 0 0 0]
      link override fft_stage_4/Mux1: xl_area=[18 36 0 36 0 0 0]
      link override fft_stage_4/butterfly/AddSub: xl_area=[12 23 0 23 0 0 0]
      link override fft_stage_4/butterfly/AddSub1: xl_area=[12 23 0 23 0 0 0]
      link override fft_stage_4/butterfly/AddSub2: xl_area=[12 23 0 23 0 0 0]
      link override fft_stage_4/butterfly/AddSub3: xl_area=[12 23 0 23 0 0 0]
      link override fft_stage_4/butterfly/Convert: xl_area=[31 18 0 61 0 0 0]
      link override fft_stage_4/butterfly/Convert1: xl_area=[31 18 0 61 0 0 0]
      link override fft_stage_4/butterfly/Convert2: xl_area=[31 18 0 61 0 0 0]
      link override fft_stage_4/butterfly/Convert3: xl_area=[31 18 0 61 0 0 0]
      link override fft_stage_4/butterfly/Delay: xl_area=[1 1 0 1 0 0 0]
      link override fft_stage_4/butterfly/Delay3: xl_area=[1 1 0 0 0 0 0]
      link override fft_stage_4/butterfly/Inverter: xl_area=[0 0 0 0 0 0 0]
      link override fft_stage_4/butterfly/Logical: xl_area=[1 1 0 1 0 0 0]
      link override fft_stage_4/butterfly/Logical1: xl_area=[1 1 0 1 0 0 0]
      link override fft_stage_4/butterfly/Logical10: xl_area=[1 1 0 1 0 0 0]
      link override fft_stage_4/butterfly/Logical11: xl_area=[1 1 0 1 0 0 0]
      link override fft_stage_4/butterfly/Logical12: xl_area=[1 1 0 1 0 0 0]
      link override fft_stage_4/butterfly/Logical13: xl_area=[1 1 0 1 0 0 0]
      link override fft_stage_4/butterfly/Logical2: xl_area=[1 1 0 1 0 0 0]
      link override fft_stage_4/butterfly/Logical3: xl_area=[1 1 0 1 0 0 0]
      link override fft_stage_4/butterfly/Logical4: xl_area=[1 1 0 1 0 0 0]
      link override fft_stage_4/butterfly/Logical5: xl_area=[1 1 0 1 0 0 0]
      link override fft_stage_4/butterfly/Logical6: xl_area=[1 1 0 1 0 0 0]
      link override fft_stage_4/butterfly/Logical7: xl_area=[1 1 0 1 0 0 0]
      link override fft_stage_4/butterfly/Logical8: xl_area=[1 1 0 1 0 0 0]
      link override fft_stage_4/butterfly/Logical9: xl_area=[1 1 0 1 0 0 0]
      link override fft_stage_4/butterfly/Mux: xl_area=[12 24 0 24 0 0 0]
      link override fft_stage_4/butterfly/Mux1: xl_area=[12 24 0 24 0 0 0]
      link override fft_stage_4/butterfly/Mux2: xl_area=[12 24 0 24 0 0 0]
      link override fft_stage_4/butterfly/Mux3: xl_area=[12 24 0 24 0 0 0]
      link override fft_stage_4/butterfly/twiddle_general/AddSub: xl_area=[11 21 0 21 0 0 0]
      link override fft_stage_4/butterfly/twiddle_general/AddSub1: xl_area=[11 21 0 21 0 0 0]
      link override fft_stage_4/butterfly/twiddle_general/Convert: xl_area=[0 0 0 0 0 0 0]
      link override fft_stage_4/butterfly/twiddle_general/Convert1: xl_area=[0 0 0 0 0 0 0]
      link override fft_stage_4/butterfly/twiddle_general/Convert2: xl_area=[0 0 0 0 0 0 0]
      link override fft_stage_4/butterfly/twiddle_general/Convert3: xl_area=[0 0 0 0 0 0 0]
      link override fft_stage_4/butterfly/twiddle_general/Delay: xl_area=[18 36 0 36 0 0 0]
      link override fft_stage_4/butterfly/twiddle_general/Delay1: xl_area=[18 36 0 0 0 0 0]
      link override fft_stage_4/butterfly/twiddle_general/Delay2: xl_area=[1 1 0 1 0 0 0]
      link override fft_stage_4/butterfly/twiddle_general/Mult: xl_area=[36 72 0 36 0 1 0]
      link override fft_stage_4/butterfly/twiddle_general/Mult1: xl_area=[36 72 0 36 0 1 0]
      link override fft_stage_4/butterfly/twiddle_general/Mult2: xl_area=[36 72 0 36 0 1 0]
      link override fft_stage_4/butterfly/twiddle_general/Mult3: xl_area=[36 72 0 36 0 1 0]
      link override fft_stage_4/butterfly/twiddle_general/br_coeff_gen/Counter: xl_area=[5 9 0 9 0 0 0]
      link override fft_stage_4/butterfly/twiddle_general/br_coeff_gen/ROM: xl_area=[9 18 0 18 0 0 0]
      link override fft_stage_4/butterfly/twiddle_general/br_coeff_gen/ROM1: xl_area=[9 18 0 17 0 0 0]
      link override fft_stage_4/butterfly/twiddle_general_3mult/AddSub: xl_area=[11 22 0 22 0 0 0]
      link override fft_stage_4/butterfly/twiddle_general_3mult/AddSub1: xl_area=[10 19 0 19 0 0 0]
      link override fft_stage_4/butterfly/twiddle_general_3mult/AddSub2: xl_area=[10 19 0 19 0 0 0]
      link override fft_stage_4/butterfly/twiddle_general_3mult/AddSub3: xl_area=[10 19 0 19 0 0 0]
      link override fft_stage_4/butterfly/twiddle_general_3mult/AddSub4: xl_area=[11 22 0 22 0 0 0]
      link override fft_stage_4/butterfly/twiddle_general_3mult/Convert: xl_area=[0 0 0 0 0 0 0]
      link override fft_stage_4/butterfly/twiddle_general_3mult/Convert1: xl_area=[0 0 0 0 0 0 0]
      link override fft_stage_4/butterfly/twiddle_general_3mult/Convert2: xl_area=[0 0 0 0 0 0 0]
      link override fft_stage_4/butterfly/twiddle_general_3mult/Convert3: xl_area=[0 0 0 0 0 0 0]
      link override fft_stage_4/butterfly/twiddle_general_3mult/Convert4: xl_area=[0 0 0 0 0 0 0]
      link override fft_stage_4/butterfly/twiddle_general_3mult/Convert5: xl_area=[0 0 0 0 0 0 0]
      link override fft_stage_4/butterfly/twiddle_general_3mult/Delay: xl_area=[18 36 0 36 0 0 0]
      link override fft_stage_4/butterfly/twiddle_general_3mult/Delay1: xl_area=[18 36 0 0 0 0 0]
      link override fft_stage_4/butterfly/twiddle_general_3mult/Delay2: xl_area=[1 1 0 1 0 0 0]
      link override fft_stage_4/butterfly/twiddle_general_3mult/Delay3: xl_area=[9 18 0 0 0 0 0]
      link override fft_stage_4/butterfly/twiddle_general_3mult/Delay4: xl_area=[9 18 0 0 0 0 0]
      link override fft_stage_4/butterfly/twiddle_general_3mult/Delay5: xl_area=[9 18 0 0 0 0 0]
      link override fft_stage_4/butterfly/twiddle_general_3mult/Mult: xl_area=[36 72 0 36 0 1 0]
      link override fft_stage_4/butterfly/twiddle_general_3mult/Mult1: xl_area=[36 72 0 36 0 1 0]
      link override fft_stage_4/butterfly/twiddle_general_3mult/Mult2: xl_area=[36 72 0 36 0 1 0]
      link override fft_stage_4/butterfly/twiddle_general_3mult/br_coeff_gen/Counter: xl_area=[5 9 0 9 0 0 0]
      link override fft_stage_4/butterfly/twiddle_general_3mult/br_coeff_gen/ROM: xl_area=[9 18 0 18 0 0 0]
      link override fft_stage_4/butterfly/twiddle_general_3mult/br_coeff_gen/ROM1: xl_area=[9 18 0 17 0 0 0]
      link override fft_stage_4/delay_b/delay_im/delay_bram/Counter: xl_area=[4 6 0 8 0 0 0]
      link override fft_stage_4/delay_b/delay_im/delay_bram/Single Port RAM: xl_area=[0 0 1 0 0 0 0]
      link override fft_stage_4/delay_b/delay_re/delay_bram/Counter: xl_area=[4 6 0 8 0 0 0]
      link override fft_stage_4/delay_b/delay_re/delay_bram/Single Port RAM: xl_area=[0 0 1 0 0 0 0]
      link override fft_stage_4/delay_b/delay_slr/delay_slr: xl_area=[72 144 0 144 0 0 0]
      link override fft_stage_4/delay_f/delay_im/delay_bram/Counter: xl_area=[4 6 0 8 0 0 0]
      link override fft_stage_4/delay_f/delay_im/delay_bram/Single Port RAM: xl_area=[0 0 1 0 0 0 0]
      link override fft_stage_4/delay_f/delay_re/delay_bram/Counter: xl_area=[4 6 0 8 0 0 0]
      link override fft_stage_4/delay_f/delay_re/delay_bram/Single Port RAM: xl_area=[0 0 1 0 0 0 0]
      link override fft_stage_4/delay_f/delay_slr/delay_slr: xl_area=[72 144 0 144 0 0 0]
      link override fft_stage_4/sync_delay_x/Counter: xl_area=[4 7 0 8 0 0 0]
      link override fft_stage_4/sync_delay_x/Logical: xl_area=[1 0 0 1 0 0 0]
      link override fft_stage_4/sync_delay_x/Mux: xl_area=[1 0 0 1 0 0 0]
      link override fft_stage_4/sync_delay_x/Relational: xl_area=[2 0 0 4 0 0 0]
      link override fft_stage_4/sync_delay_x/Relational1: xl_area=[2 0 0 4 0 0 0]
      link override fft_stage_5/Counter: xl_area=[3 6 0 6 0 0 0]
      link override fft_stage_5/Delay: xl_area=[1 1 0 0 0 0 0]
      link override fft_stage_5/Logical1: xl_area=[1 1 0 1 0 0 0]
      link override fft_stage_5/Mux: xl_area=[18 36 0 36 0 0 0]
      link override fft_stage_5/Mux1: xl_area=[18 36 0 36 0 0 0]
      link override fft_stage_5/butterfly/AddSub: xl_area=[12 23 0 23 0 0 0]
      link override fft_stage_5/butterfly/AddSub1: xl_area=[12 23 0 23 0 0 0]
      link override fft_stage_5/butterfly/AddSub2: xl_area=[12 23 0 23 0 0 0]
      link override fft_stage_5/butterfly/AddSub3: xl_area=[12 23 0 23 0 0 0]
      link override fft_stage_5/butterfly/Convert: xl_area=[31 18 0 61 0 0 0]
      link override fft_stage_5/butterfly/Convert1: xl_area=[31 18 0 61 0 0 0]
      link override fft_stage_5/butterfly/Convert2: xl_area=[31 18 0 61 0 0 0]
      link override fft_stage_5/butterfly/Convert3: xl_area=[31 18 0 61 0 0 0]
      link override fft_stage_5/butterfly/Delay: xl_area=[1 1 0 1 0 0 0]
      link override fft_stage_5/butterfly/Delay3: xl_area=[1 1 0 0 0 0 0]
      link override fft_stage_5/butterfly/Inverter: xl_area=[0 0 0 0 0 0 0]
      link override fft_stage_5/butterfly/Logical: xl_area=[1 1 0 1 0 0 0]
      link override fft_stage_5/butterfly/Logical1: xl_area=[1 1 0 1 0 0 0]
      link override fft_stage_5/butterfly/Logical10: xl_area=[1 1 0 1 0 0 0]
      link override fft_stage_5/butterfly/Logical11: xl_area=[1 1 0 1 0 0 0]
      link override fft_stage_5/butterfly/Logical12: xl_area=[1 1 0 1 0 0 0]
      link override fft_stage_5/butterfly/Logical13: xl_area=[1 1 0 1 0 0 0]
      link override fft_stage_5/butterfly/Logical2: xl_area=[1 1 0 1 0 0 0]
      link override fft_stage_5/butterfly/Logical3: xl_area=[1 1 0 1 0 0 0]
      link override fft_stage_5/butterfly/Logical4: xl_area=[1 1 0 1 0 0 0]
      link override fft_stage_5/butterfly/Logical5: xl_area=[1 1 0 1 0 0 0]
      link override fft_stage_5/butterfly/Logical6: xl_area=[1 1 0 1 0 0 0]
      link override fft_stage_5/butterfly/Logical7: xl_area=[1 1 0 1 0 0 0]
      link override fft_stage_5/butterfly/Logical8: xl_area=[1 1 0 1 0 0 0]
      link override fft_stage_5/butterfly/Logical9: xl_area=[1 1 0 1 0 0 0]
      link override fft_stage_5/butterfly/Mux: xl_area=[12 24 0 24 0 0 0]
      link override fft_stage_5/butterfly/Mux1: xl_area=[12 24 0 24 0 0 0]
      link override fft_stage_5/butterfly/Mux2: xl_area=[12 24 0 24 0 0 0]
      link override fft_stage_5/butterfly/Mux3: xl_area=[12 24 0 24 0 0 0]
      link override fft_stage_5/butterfly/twiddle_general/AddSub: xl_area=[11 21 0 21 0 0 0]
      link override fft_stage_5/butterfly/twiddle_general/AddSub1: xl_area=[11 21 0 21 0 0 0]
      link override fft_stage_5/butterfly/twiddle_general/Convert: xl_area=[0 0 0 0 0 0 0]
      link override fft_stage_5/butterfly/twiddle_general/Convert1: xl_area=[0 0 0 0 0 0 0]
      link override fft_stage_5/butterfly/twiddle_general/Convert2: xl_area=[0 0 0 0 0 0 0]
      link override fft_stage_5/butterfly/twiddle_general/Convert3: xl_area=[0 0 0 0 0 0 0]
      link override fft_stage_5/butterfly/twiddle_general/Delay: xl_area=[18 36 0 36 0 0 0]
      link override fft_stage_5/butterfly/twiddle_general/Delay1: xl_area=[18 36 0 0 0 0 0]
      link override fft_stage_5/butterfly/twiddle_general/Delay2: xl_area=[1 1 0 1 0 0 0]
      link override fft_stage_5/butterfly/twiddle_general/Mult: xl_area=[36 72 0 36 0 1 0]
      link override fft_stage_5/butterfly/twiddle_general/Mult1: xl_area=[36 72 0 36 0 1 0]
      link override fft_stage_5/butterfly/twiddle_general/Mult2: xl_area=[36 72 0 36 0 1 0]
      link override fft_stage_5/butterfly/twiddle_general/Mult3: xl_area=[36 72 0 36 0 1 0]
      link override fft_stage_5/butterfly/twiddle_general/br_coeff_gen/Counter: xl_area=[5 9 0 9 0 0 0]
      link override fft_stage_5/butterfly/twiddle_general/br_coeff_gen/ROM: xl_area=[9 18 0 18 0 0 0]
      link override fft_stage_5/butterfly/twiddle_general/br_coeff_gen/ROM1: xl_area=[9 18 0 18 0 0 0]
      link override fft_stage_5/butterfly/twiddle_general_3mult/AddSub: xl_area=[11 22 0 22 0 0 0]
      link override fft_stage_5/butterfly/twiddle_general_3mult/AddSub1: xl_area=[10 19 0 19 0 0 0]
      link override fft_stage_5/butterfly/twiddle_general_3mult/AddSub2: xl_area=[10 19 0 19 0 0 0]
      link override fft_stage_5/butterfly/twiddle_general_3mult/AddSub3: xl_area=[10 19 0 19 0 0 0]
      link override fft_stage_5/butterfly/twiddle_general_3mult/AddSub4: xl_area=[11 22 0 22 0 0 0]
      link override fft_stage_5/butterfly/twiddle_general_3mult/Convert: xl_area=[0 0 0 0 0 0 0]
      link override fft_stage_5/butterfly/twiddle_general_3mult/Convert1: xl_area=[0 0 0 0 0 0 0]
      link override fft_stage_5/butterfly/twiddle_general_3mult/Convert2: xl_area=[0 0 0 0 0 0 0]
      link override fft_stage_5/butterfly/twiddle_general_3mult/Convert3: xl_area=[0 0 0 0 0 0 0]
      link override fft_stage_5/butterfly/twiddle_general_3mult/Convert4: xl_area=[0 0 0 0 0 0 0]
      link override fft_stage_5/butterfly/twiddle_general_3mult/Convert5: xl_area=[0 0 0 0 0 0 0]
      link override fft_stage_5/butterfly/twiddle_general_3mult/Delay: xl_area=[18 36 0 36 0 0 0]
      link override fft_stage_5/butterfly/twiddle_general_3mult/Delay1: xl_area=[18 36 0 0 0 0 0]
      link override fft_stage_5/butterfly/twiddle_general_3mult/Delay2: xl_area=[1 1 0 1 0 0 0]
      link override fft_stage_5/butterfly/twiddle_general_3mult/Delay3: xl_area=[9 18 0 0 0 0 0]
      link override fft_stage_5/butterfly/twiddle_general_3mult/Delay4: xl_area=[9 18 0 0 0 0 0]
      link override fft_stage_5/butterfly/twiddle_general_3mult/Delay5: xl_area=[9 18 0 0 0 0 0]
      link override fft_stage_5/butterfly/twiddle_general_3mult/Mult: xl_area=[36 72 0 36 0 1 0]
      link override fft_stage_5/butterfly/twiddle_general_3mult/Mult1: xl_area=[36 72 0 36 0 1 0]
      link override fft_stage_5/butterfly/twiddle_general_3mult/Mult2: xl_area=[36 72 0 36 0 1 0]
      link override fft_stage_5/butterfly/twiddle_general_3mult/br_coeff_gen/Counter: xl_area=[5 9 0 9 0 0 0]
      link override fft_stage_5/butterfly/twiddle_general_3mult/br_coeff_gen/ROM: xl_area=[9 18 0 18 0 0 0]
      link override fft_stage_5/butterfly/twiddle_general_3mult/br_coeff_gen/ROM1: xl_area=[9 18 0 18 0 0 0]
      link override fft_stage_5/delay_b/delay_im/delay_slr/delay_slr: xl_area=[18 36 0 36 0 0 0]
      link override fft_stage_5/delay_b/delay_re/delay_slr/delay_slr: xl_area=[18 36 0 36 0 0 0]
      link override fft_stage_5/delay_b/delay_slr/delay_slr: xl_area=[36 72 0 72 0 0 0]
      link override fft_stage_5/delay_f/delay_im/delay_slr/delay_slr: xl_area=[18 36 0 36 0 0 0]
      link override fft_stage_5/delay_f/delay_re/delay_slr/delay_slr: xl_area=[18 36 0 36 0 0 0]
      link override fft_stage_5/delay_f/delay_slr/delay_slr: xl_area=[36 72 0 72 0 0 0]
      link override fft_stage_5/sync_delay_x/Counter: xl_area=[4 6 0 7 0 0 0]
      link override fft_stage_5/sync_delay_x/Logical: xl_area=[1 0 0 1 0 0 0]
      link override fft_stage_5/sync_delay_x/Mux: xl_area=[1 0 0 1 0 0 0]
      link override fft_stage_5/sync_delay_x/Relational: xl_area=[2 0 0 3 0 0 0]
      link override fft_stage_5/sync_delay_x/Relational1: xl_area=[2 0 0 3 0 0 0]
      link override fft_stage_6/Counter: xl_area=[3 5 0 5 0 0 0]
      link override fft_stage_6/Delay: xl_area=[1 1 0 0 0 0 0]
      link override fft_stage_6/Logical1: xl_area=[1 1 0 1 0 0 0]
      link override fft_stage_6/Mux: xl_area=[18 36 0 36 0 0 0]
      link override fft_stage_6/Mux1: xl_area=[18 36 0 36 0 0 0]
      link override fft_stage_6/butterfly/AddSub: xl_area=[12 23 0 23 0 0 0]
      link override fft_stage_6/butterfly/AddSub1: xl_area=[12 23 0 23 0 0 0]
      link override fft_stage_6/butterfly/AddSub2: xl_area=[12 23 0 23 0 0 0]
      link override fft_stage_6/butterfly/AddSub3: xl_area=[12 23 0 23 0 0 0]
      link override fft_stage_6/butterfly/Convert: xl_area=[31 18 0 61 0 0 0]
      link override fft_stage_6/butterfly/Convert1: xl_area=[31 18 0 61 0 0 0]
      link override fft_stage_6/butterfly/Convert2: xl_area=[31 18 0 61 0 0 0]
      link override fft_stage_6/butterfly/Convert3: xl_area=[31 18 0 61 0 0 0]
      link override fft_stage_6/butterfly/Delay: xl_area=[1 1 0 1 0 0 0]
      link override fft_stage_6/butterfly/Delay3: xl_area=[1 1 0 0 0 0 0]
      link override fft_stage_6/butterfly/Inverter: xl_area=[0 0 0 0 0 0 0]
      link override fft_stage_6/butterfly/Logical: xl_area=[1 1 0 1 0 0 0]
      link override fft_stage_6/butterfly/Logical1: xl_area=[1 1 0 1 0 0 0]
      link override fft_stage_6/butterfly/Logical10: xl_area=[1 1 0 1 0 0 0]
      link override fft_stage_6/butterfly/Logical11: xl_area=[1 1 0 1 0 0 0]
      link override fft_stage_6/butterfly/Logical12: xl_area=[1 1 0 1 0 0 0]
      link override fft_stage_6/butterfly/Logical13: xl_area=[1 1 0 1 0 0 0]
      link override fft_stage_6/butterfly/Logical2: xl_area=[1 1 0 1 0 0 0]
      link override fft_stage_6/butterfly/Logical3: xl_area=[1 1 0 1 0 0 0]
      link override fft_stage_6/butterfly/Logical4: xl_area=[1 1 0 1 0 0 0]
      link override fft_stage_6/butterfly/Logical5: xl_area=[1 1 0 1 0 0 0]
      link override fft_stage_6/butterfly/Logical6: xl_area=[1 1 0 1 0 0 0]
      link override fft_stage_6/butterfly/Logical7: xl_area=[1 1 0 1 0 0 0]
      link override fft_stage_6/butterfly/Logical8: xl_area=[1 1 0 1 0 0 0]
      link override fft_stage_6/butterfly/Logical9: xl_area=[1 1 0 1 0 0 0]
      link override fft_stage_6/butterfly/Mux: xl_area=[12 24 0 24 0 0 0]
      link override fft_stage_6/butterfly/Mux1: xl_area=[12 24 0 24 0 0 0]
      link override fft_stage_6/butterfly/Mux2: xl_area=[12 24 0 24 0 0 0]
      link override fft_stage_6/butterfly/Mux3: xl_area=[12 24 0 24 0 0 0]
      link override fft_stage_6/butterfly/twiddle_general/AddSub: xl_area=[11 21 0 21 0 0 0]
      link override fft_stage_6/butterfly/twiddle_general/AddSub1: xl_area=[11 21 0 21 0 0 0]
      link override fft_stage_6/butterfly/twiddle_general/Convert: xl_area=[0 0 0 0 0 0 0]
      link override fft_stage_6/butterfly/twiddle_general/Convert1: xl_area=[0 0 0 0 0 0 0]
      link override fft_stage_6/butterfly/twiddle_general/Convert2: xl_area=[0 0 0 0 0 0 0]
      link override fft_stage_6/butterfly/twiddle_general/Convert3: xl_area=[0 0 0 0 0 0 0]
      link override fft_stage_6/butterfly/twiddle_general/Delay: xl_area=[18 36 0 36 0 0 0]
      link override fft_stage_6/butterfly/twiddle_general/Delay1: xl_area=[18 36 0 0 0 0 0]
      link override fft_stage_6/butterfly/twiddle_general/Delay2: xl_area=[1 1 0 1 0 0 0]
      link override fft_stage_6/butterfly/twiddle_general/Mult: xl_area=[36 72 0 36 0 1 0]
      link override fft_stage_6/butterfly/twiddle_general/Mult1: xl_area=[36 72 0 36 0 1 0]
      link override fft_stage_6/butterfly/twiddle_general/Mult2: xl_area=[36 72 0 36 0 1 0]
      link override fft_stage_6/butterfly/twiddle_general/Mult3: xl_area=[36 72 0 36 0 1 0]
      link override fft_stage_6/butterfly/twiddle_general/br_coeff_gen/Counter: xl_area=[5 9 0 9 0 0 0]
      link override fft_stage_6/butterfly/twiddle_general/br_coeff_gen/ROM: xl_area=[18 18 0 36 0 0 0]
      link override fft_stage_6/butterfly/twiddle_general/br_coeff_gen/ROM1: xl_area=[18 18 0 35 0 0 0]
      link override fft_stage_6/butterfly/twiddle_general_3mult/AddSub: xl_area=[11 22 0 22 0 0 0]
      link override fft_stage_6/butterfly/twiddle_general_3mult/AddSub1: xl_area=[10 19 0 19 0 0 0]
      link override fft_stage_6/butterfly/twiddle_general_3mult/AddSub2: xl_area=[10 19 0 19 0 0 0]
      link override fft_stage_6/butterfly/twiddle_general_3mult/AddSub3: xl_area=[10 19 0 19 0 0 0]
      link override fft_stage_6/butterfly/twiddle_general_3mult/AddSub4: xl_area=[11 22 0 22 0 0 0]
      link override fft_stage_6/butterfly/twiddle_general_3mult/Convert: xl_area=[0 0 0 0 0 0 0]
      link override fft_stage_6/butterfly/twiddle_general_3mult/Convert1: xl_area=[0 0 0 0 0 0 0]
      link override fft_stage_6/butterfly/twiddle_general_3mult/Convert2: xl_area=[0 0 0 0 0 0 0]
      link override fft_stage_6/butterfly/twiddle_general_3mult/Convert3: xl_area=[0 0 0 0 0 0 0]
      link override fft_stage_6/butterfly/twiddle_general_3mult/Convert4: xl_area=[0 0 0 0 0 0 0]
      link override fft_stage_6/butterfly/twiddle_general_3mult/Convert5: xl_area=[0 0 0 0 0 0 0]
      link override fft_stage_6/butterfly/twiddle_general_3mult/Delay: xl_area=[18 36 0 36 0 0 0]
      link override fft_stage_6/butterfly/twiddle_general_3mult/Delay1: xl_area=[18 36 0 0 0 0 0]
      link override fft_stage_6/butterfly/twiddle_general_3mult/Delay2: xl_area=[1 1 0 1 0 0 0]
      link override fft_stage_6/butterfly/twiddle_general_3mult/Delay3: xl_area=[9 18 0 0 0 0 0]
      link override fft_stage_6/butterfly/twiddle_general_3mult/Delay4: xl_area=[9 18 0 0 0 0 0]
      link override fft_stage_6/butterfly/twiddle_general_3mult/Delay5: xl_area=[9 18 0 0 0 0 0]
      link override fft_stage_6/butterfly/twiddle_general_3mult/Mult: xl_area=[36 72 0 36 0 1 0]
      link override fft_stage_6/butterfly/twiddle_general_3mult/Mult1: xl_area=[36 72 0 36 0 1 0]
      link override fft_stage_6/butterfly/twiddle_general_3mult/Mult2: xl_area=[36 72 0 36 0 1 0]
      link override fft_stage_6/butterfly/twiddle_general_3mult/br_coeff_gen/Counter: xl_area=[5 9 0 9 0 0 0]
      link override fft_stage_6/butterfly/twiddle_general_3mult/br_coeff_gen/ROM: xl_area=[18 18 0 36 0 0 0]
      link override fft_stage_6/butterfly/twiddle_general_3mult/br_coeff_gen/ROM1: xl_area=[18 18 0 35 0 0 0]
      link override fft_stage_6/delay_b/delay_im/delay_slr/delay_slr: xl_area=[9 18 0 18 0 0 0]
      link override fft_stage_6/delay_b/delay_re/delay_slr/delay_slr: xl_area=[9 18 0 18 0 0 0]
      link override fft_stage_6/delay_b/delay_slr/delay_slr: xl_area=[18 36 0 36 0 0 0]
      link override fft_stage_6/delay_f/delay_im/delay_slr/delay_slr: xl_area=[9 18 0 18 0 0 0]
      link override fft_stage_6/delay_f/delay_re/delay_slr/delay_slr: xl_area=[9 18 0 18 0 0 0]
      link override fft_stage_6/delay_f/delay_slr/delay_slr: xl_area=[18 36 0 36 0 0 0]
      link override fft_stage_6/sync_delay_x/Counter: xl_area=[3 5 0 6 0 0 0]
      link override fft_stage_6/sync_delay_x/Logical: xl_area=[1 0 0 1 0 0 0]
      link override fft_stage_6/sync_delay_x/Mux: xl_area=[1 0 0 1 0 0 0]
      link override fft_stage_6/sync_delay_x/Relational: xl_area=[2 0 0 3 0 0 0]
      link override fft_stage_6/sync_delay_x/Relational1: xl_area=[2 0 0 3 0 0 0]
      link override fft_stage_7/Counter: xl_area=[2 4 0 4 0 0 0]
      link override fft_stage_7/Delay: xl_area=[1 1 0 0 0 0 0]
      link override fft_stage_7/Logical1: xl_area=[1 1 0 1 0 0 0]
      link override fft_stage_7/Mux: xl_area=[18 36 0 36 0 0 0]
      link override fft_stage_7/Mux1: xl_area=[18 36 0 36 0 0 0]
      link override fft_stage_7/butterfly/AddSub: xl_area=[12 23 0 23 0 0 0]
      link override fft_stage_7/butterfly/AddSub1: xl_area=[12 23 0 23 0 0 0]
      link override fft_stage_7/butterfly/AddSub2: xl_area=[12 23 0 23 0 0 0]
      link override fft_stage_7/butterfly/AddSub3: xl_area=[12 23 0 23 0 0 0]
      link override fft_stage_7/butterfly/Convert: xl_area=[31 18 0 61 0 0 0]
      link override fft_stage_7/butterfly/Convert1: xl_area=[31 18 0 61 0 0 0]
      link override fft_stage_7/butterfly/Convert2: xl_area=[31 18 0 61 0 0 0]
      link override fft_stage_7/butterfly/Convert3: xl_area=[31 18 0 61 0 0 0]
      link override fft_stage_7/butterfly/Delay: xl_area=[1 1 0 1 0 0 0]
      link override fft_stage_7/butterfly/Delay3: xl_area=[1 1 0 0 0 0 0]
      link override fft_stage_7/butterfly/Inverter: xl_area=[0 0 0 0 0 0 0]
      link override fft_stage_7/butterfly/Logical: xl_area=[1 1 0 1 0 0 0]
      link override fft_stage_7/butterfly/Logical1: xl_area=[1 1 0 1 0 0 0]
      link override fft_stage_7/butterfly/Logical10: xl_area=[1 1 0 1 0 0 0]
      link override fft_stage_7/butterfly/Logical11: xl_area=[1 1 0 1 0 0 0]
      link override fft_stage_7/butterfly/Logical12: xl_area=[1 1 0 1 0 0 0]
      link override fft_stage_7/butterfly/Logical13: xl_area=[1 1 0 1 0 0 0]
      link override fft_stage_7/butterfly/Logical2: xl_area=[1 1 0 1 0 0 0]
      link override fft_stage_7/butterfly/Logical3: xl_area=[1 1 0 1 0 0 0]
      link override fft_stage_7/butterfly/Logical4: xl_area=[1 1 0 1 0 0 0]
      link override fft_stage_7/butterfly/Logical5: xl_area=[1 1 0 1 0 0 0]
      link override fft_stage_7/butterfly/Logical6: xl_area=[1 1 0 1 0 0 0]
      link override fft_stage_7/butterfly/Logical7: xl_area=[1 1 0 1 0 0 0]
      link override fft_stage_7/butterfly/Logical8: xl_area=[1 1 0 1 0 0 0]
      link override fft_stage_7/butterfly/Logical9: xl_area=[1 1 0 1 0 0 0]
      link override fft_stage_7/butterfly/Mux: xl_area=[12 24 0 24 0 0 0]
      link override fft_stage_7/butterfly/Mux1: xl_area=[12 24 0 24 0 0 0]
      link override fft_stage_7/butterfly/Mux2: xl_area=[12 24 0 24 0 0 0]
      link override fft_stage_7/butterfly/Mux3: xl_area=[12 24 0 24 0 0 0]
      link override fft_stage_7/butterfly/twiddle_general/AddSub: xl_area=[11 21 0 21 0 0 0]
      link override fft_stage_7/butterfly/twiddle_general/AddSub1: xl_area=[11 21 0 21 0 0 0]
      link override fft_stage_7/butterfly/twiddle_general/Convert: xl_area=[0 0 0 0 0 0 0]
      link override fft_stage_7/butterfly/twiddle_general/Convert1: xl_area=[0 0 0 0 0 0 0]
      link override fft_stage_7/butterfly/twiddle_general/Convert2: xl_area=[0 0 0 0 0 0 0]
      link override fft_stage_7/butterfly/twiddle_general/Convert3: xl_area=[0 0 0 0 0 0 0]
      link override fft_stage_7/butterfly/twiddle_general/Delay: xl_area=[18 36 0 36 0 0 0]
      link override fft_stage_7/butterfly/twiddle_general/Delay1: xl_area=[18 36 0 0 0 0 0]
      link override fft_stage_7/butterfly/twiddle_general/Delay2: xl_area=[1 1 0 1 0 0 0]
      link override fft_stage_7/butterfly/twiddle_general/Mult: xl_area=[36 72 0 36 0 1 0]
      link override fft_stage_7/butterfly/twiddle_general/Mult1: xl_area=[36 72 0 36 0 1 0]
      link override fft_stage_7/butterfly/twiddle_general/Mult2: xl_area=[36 72 0 36 0 1 0]
      link override fft_stage_7/butterfly/twiddle_general/Mult3: xl_area=[36 72 0 36 0 1 0]
      link override fft_stage_7/butterfly/twiddle_general/br_coeff_gen/Counter: xl_area=[5 9 0 9 0 0 0]
      link override fft_stage_7/butterfly/twiddle_general/br_coeff_gen/ROM: xl_area=[36 18 0 72 0 0 0]
      link override fft_stage_7/butterfly/twiddle_general/br_coeff_gen/ROM1: xl_area=[35 18 0 69 0 0 0]
      link override fft_stage_7/butterfly/twiddle_general_3mult/AddSub: xl_area=[11 22 0 22 0 0 0]
      link override fft_stage_7/butterfly/twiddle_general_3mult/AddSub1: xl_area=[10 19 0 19 0 0 0]
      link override fft_stage_7/butterfly/twiddle_general_3mult/AddSub2: xl_area=[10 19 0 19 0 0 0]
      link override fft_stage_7/butterfly/twiddle_general_3mult/AddSub3: xl_area=[10 19 0 19 0 0 0]
      link override fft_stage_7/butterfly/twiddle_general_3mult/AddSub4: xl_area=[11 22 0 22 0 0 0]
      link override fft_stage_7/butterfly/twiddle_general_3mult/Convert: xl_area=[0 0 0 0 0 0 0]
      link override fft_stage_7/butterfly/twiddle_general_3mult/Convert1: xl_area=[0 0 0 0 0 0 0]
      link override fft_stage_7/butterfly/twiddle_general_3mult/Convert2: xl_area=[0 0 0 0 0 0 0]
      link override fft_stage_7/butterfly/twiddle_general_3mult/Convert3: xl_area=[0 0 0 0 0 0 0]
      link override fft_stage_7/butterfly/twiddle_general_3mult/Convert4: xl_area=[0 0 0 0 0 0 0]
      link override fft_stage_7/butterfly/twiddle_general_3mult/Convert5: xl_area=[0 0 0 0 0 0 0]
      link override fft_stage_7/butterfly/twiddle_general_3mult/Delay: xl_area=[18 36 0 36 0 0 0]
      link override fft_stage_7/butterfly/twiddle_general_3mult/Delay1: xl_area=[18 36 0 0 0 0 0]
      link override fft_stage_7/butterfly/twiddle_general_3mult/Delay2: xl_area=[1 1 0 1 0 0 0]
      link override fft_stage_7/butterfly/twiddle_general_3mult/Delay3: xl_area=[9 18 0 0 0 0 0]
      link override fft_stage_7/butterfly/twiddle_general_3mult/Delay4: xl_area=[9 18 0 0 0 0 0]
      link override fft_stage_7/butterfly/twiddle_general_3mult/Delay5: xl_area=[9 18 0 0 0 0 0]
      link override fft_stage_7/butterfly/twiddle_general_3mult/Mult: xl_area=[36 72 0 36 0 1 0]
      link override fft_stage_7/butterfly/twiddle_general_3mult/Mult1: xl_area=[36 72 0 36 0 1 0]
      link override fft_stage_7/butterfly/twiddle_general_3mult/Mult2: xl_area=[36 72 0 36 0 1 0]
      link override fft_stage_7/butterfly/twiddle_general_3mult/br_coeff_gen/Counter: xl_area=[5 9 0 9 0 0 0]
      link override fft_stage_7/butterfly/twiddle_general_3mult/br_coeff_gen/ROM: xl_area=[36 18 0 72 0 0 0]
      link override fft_stage_7/butterfly/twiddle_general_3mult/br_coeff_gen/ROM1: xl_area=[35 18 0 69 0 0 0]
      link override fft_stage_7/delay_b/delay_im/delay_slr/delay_slr: xl_area=[9 18 0 18 0 0 0]
      link override fft_stage_7/delay_b/delay_re/delay_slr/delay_slr: xl_area=[9 18 0 18 0 0 0]
      link override fft_stage_7/delay_b/delay_slr/delay_slr: xl_area=[18 36 0 36 0 0 0]
      link override fft_stage_7/delay_f/delay_im/delay_slr/delay_slr: xl_area=[9 18 0 18 0 0 0]
      link override fft_stage_7/delay_f/delay_re/delay_slr/delay_slr: xl_area=[9 18 0 18 0 0 0]
      link override fft_stage_7/delay_f/delay_slr/delay_slr: xl_area=[18 36 0 36 0 0 0]
      link override fft_stage_7/sync_delay_x/Counter: xl_area=[3 4 0 5 0 0 0]
      link override fft_stage_7/sync_delay_x/Logical: xl_area=[1 0 0 1 0 0 0]
      link override fft_stage_7/sync_delay_x/Mux: xl_area=[1 0 0 1 0 0 0]
      link override fft_stage_7/sync_delay_x/Relational: xl_area=[1 0 0 2 0 0 0]
      link override fft_stage_7/sync_delay_x/Relational1: xl_area=[1 0 0 2 0 0 0]
      link override fft_stage_8/Counter: xl_area=[2 3 0 3 0 0 0]
      link override fft_stage_8/Delay: xl_area=[1 1 0 0 0 0 0]
      link override fft_stage_8/Logical1: xl_area=[1 1 0 1 0 0 0]
      link override fft_stage_8/Mux: xl_area=[18 36 0 36 0 0 0]
      link override fft_stage_8/Mux1: xl_area=[18 36 0 36 0 0 0]
      link override fft_stage_8/butterfly/AddSub: xl_area=[12 23 0 23 0 0 0]
      link override fft_stage_8/butterfly/AddSub1: xl_area=[12 23 0 23 0 0 0]
      link override fft_stage_8/butterfly/AddSub2: xl_area=[12 23 0 23 0 0 0]
      link override fft_stage_8/butterfly/AddSub3: xl_area=[12 23 0 23 0 0 0]
      link override fft_stage_8/butterfly/Convert: xl_area=[31 18 0 61 0 0 0]
      link override fft_stage_8/butterfly/Convert1: xl_area=[31 18 0 61 0 0 0]
      link override fft_stage_8/butterfly/Convert2: xl_area=[31 18 0 61 0 0 0]
      link override fft_stage_8/butterfly/Convert3: xl_area=[31 18 0 61 0 0 0]
      link override fft_stage_8/butterfly/Delay: xl_area=[1 1 0 1 0 0 0]
      link override fft_stage_8/butterfly/Delay3: xl_area=[1 1 0 0 0 0 0]
      link override fft_stage_8/butterfly/Inverter: xl_area=[0 0 0 0 0 0 0]
      link override fft_stage_8/butterfly/Logical: xl_area=[1 1 0 1 0 0 0]
      link override fft_stage_8/butterfly/Logical1: xl_area=[1 1 0 1 0 0 0]
      link override fft_stage_8/butterfly/Logical10: xl_area=[1 1 0 1 0 0 0]
      link override fft_stage_8/butterfly/Logical11: xl_area=[1 1 0 1 0 0 0]
      link override fft_stage_8/butterfly/Logical12: xl_area=[1 1 0 1 0 0 0]
      link override fft_stage_8/butterfly/Logical13: xl_area=[1 1 0 1 0 0 0]
      link override fft_stage_8/butterfly/Logical2: xl_area=[1 1 0 1 0 0 0]
      link override fft_stage_8/butterfly/Logical3: xl_area=[1 1 0 1 0 0 0]
      link override fft_stage_8/butterfly/Logical4: xl_area=[1 1 0 1 0 0 0]
      link override fft_stage_8/butterfly/Logical5: xl_area=[1 1 0 1 0 0 0]
      link override fft_stage_8/butterfly/Logical6: xl_area=[1 1 0 1 0 0 0]
      link override fft_stage_8/butterfly/Logical7: xl_area=[1 1 0 1 0 0 0]
      link override fft_stage_8/butterfly/Logical8: xl_area=[1 1 0 1 0 0 0]
      link override fft_stage_8/butterfly/Logical9: xl_area=[1 1 0 1 0 0 0]
      link override fft_stage_8/butterfly/Mux: xl_area=[12 24 0 24 0 0 0]
      link override fft_stage_8/butterfly/Mux1: xl_area=[12 24 0 24 0 0 0]
      link override fft_stage_8/butterfly/Mux2: xl_area=[12 24 0 24 0 0 0]
      link override fft_stage_8/butterfly/Mux3: xl_area=[12 24 0 24 0 0 0]
      link override fft_stage_8/butterfly/twiddle_general/AddSub: xl_area=[11 21 0 21 0 0 0]
      link override fft_stage_8/butterfly/twiddle_general/AddSub1: xl_area=[11 21 0 21 0 0 0]
      link override fft_stage_8/butterfly/twiddle_general/Convert: xl_area=[0 0 0 0 0 0 0]
      link override fft_stage_8/butterfly/twiddle_general/Convert1: xl_area=[0 0 0 0 0 0 0]
      link override fft_stage_8/butterfly/twiddle_general/Convert2: xl_area=[0 0 0 0 0 0 0]
      link override fft_stage_8/butterfly/twiddle_general/Convert3: xl_area=[0 0 0 0 0 0 0]
      link override fft_stage_8/butterfly/twiddle_general/Delay: xl_area=[18 36 0 36 0 0 0]
      link override fft_stage_8/butterfly/twiddle_general/Delay1: xl_area=[18 36 0 0 0 0 0]
      link override fft_stage_8/butterfly/twiddle_general/Delay2: xl_area=[1 1 0 1 0 0 0]
      link override fft_stage_8/butterfly/twiddle_general/Mult: xl_area=[36 72 0 36 0 1 0]
      link override fft_stage_8/butterfly/twiddle_general/Mult1: xl_area=[36 72 0 36 0 1 0]
      link override fft_stage_8/butterfly/twiddle_general/Mult2: xl_area=[36 72 0 36 0 1 0]
      link override fft_stage_8/butterfly/twiddle_general/Mult3: xl_area=[36 72 0 36 0 1 0]
      link override fft_stage_8/butterfly/twiddle_general/br_coeff_gen/Counter: xl_area=[5 9 0 9 0 0 0]
      link override fft_stage_8/butterfly/twiddle_general/br_coeff_gen/ROM: xl_area=[72 18 0 144 0 0 0]
      link override fft_stage_8/butterfly/twiddle_general/br_coeff_gen/ROM1: xl_area=[69 18 0 137 0 0 0]
      link override fft_stage_8/butterfly/twiddle_general_3mult/AddSub: xl_area=[11 22 0 22 0 0 0]
      link override fft_stage_8/butterfly/twiddle_general_3mult/AddSub1: xl_area=[10 19 0 19 0 0 0]
      link override fft_stage_8/butterfly/twiddle_general_3mult/AddSub2: xl_area=[10 19 0 19 0 0 0]
      link override fft_stage_8/butterfly/twiddle_general_3mult/AddSub3: xl_area=[10 19 0 19 0 0 0]
      link override fft_stage_8/butterfly/twiddle_general_3mult/AddSub4: xl_area=[11 22 0 22 0 0 0]
      link override fft_stage_8/butterfly/twiddle_general_3mult/Convert: xl_area=[0 0 0 0 0 0 0]
      link override fft_stage_8/butterfly/twiddle_general_3mult/Convert1: xl_area=[0 0 0 0 0 0 0]
      link override fft_stage_8/butterfly/twiddle_general_3mult/Convert2: xl_area=[0 0 0 0 0 0 0]
      link override fft_stage_8/butterfly/twiddle_general_3mult/Convert3: xl_area=[0 0 0 0 0 0 0]
      link override fft_stage_8/butterfly/twiddle_general_3mult/Convert4: xl_area=[0 0 0 0 0 0 0]
      link override fft_stage_8/butterfly/twiddle_general_3mult/Convert5: xl_area=[0 0 0 0 0 0 0]
      link override fft_stage_8/butterfly/twiddle_general_3mult/Delay: xl_area=[18 36 0 36 0 0 0]
      link override fft_stage_8/butterfly/twiddle_general_3mult/Delay1: xl_area=[18 36 0 0 0 0 0]
      link override fft_stage_8/butterfly/twiddle_general_3mult/Delay2: xl_area=[1 1 0 1 0 0 0]
      link override fft_stage_8/butterfly/twiddle_general_3mult/Delay3: xl_area=[9 18 0 0 0 0 0]
      link override fft_stage_8/butterfly/twiddle_general_3mult/Delay4: xl_area=[9 18 0 0 0 0 0]
      link override fft_stage_8/butterfly/twiddle_general_3mult/Delay5: xl_area=[9 18 0 0 0 0 0]
      link override fft_stage_8/butterfly/twiddle_general_3mult/Mult: xl_area=[36 72 0 36 0 1 0]
      link override fft_stage_8/butterfly/twiddle_general_3mult/Mult1: xl_area=[36 72 0 36 0 1 0]
      link override fft_stage_8/butterfly/twiddle_general_3mult/Mult2: xl_area=[36 72 0 36 0 1 0]
      link override fft_stage_8/butterfly/twiddle_general_3mult/br_coeff_gen/Counter: xl_area=[5 9 0 9 0 0 0]
      link override fft_stage_8/butterfly/twiddle_general_3mult/br_coeff_gen/ROM: xl_area=[72 18 0 144 0 0 0]
      link override fft_stage_8/butterfly/twiddle_general_3mult/br_coeff_gen/ROM1: xl_area=[69 18 0 137 0 0 0]
      link override fft_stage_8/delay_b/delay_im/delay_slr/delay_slr: xl_area=[9 18 0 18 0 0 0]
      link override fft_stage_8/delay_b/delay_re/delay_slr/delay_slr: xl_area=[9 18 0 18 0 0 0]
      link override fft_stage_8/delay_b/delay_slr/delay_slr: xl_area=[18 36 0 36 0 0 0]
      link override fft_stage_8/delay_f/delay_im/delay_slr/delay_slr: xl_area=[9 18 0 18 0 0 0]
      link override fft_stage_8/delay_f/delay_re/delay_slr/delay_slr: xl_area=[9 18 0 18 0 0 0]
      link override fft_stage_8/delay_f/delay_slr/delay_slr: xl_area=[18 36 0 36 0 0 0]
      link override fft_stage_8/sync_delay_x/Counter: xl_area=[2 3 0 4 0 0 0]
      link override fft_stage_8/sync_delay_x/Logical: xl_area=[1 0 0 1 0 0 0]
      link override fft_stage_8/sync_delay_x/Mux: xl_area=[1 0 0 1 0 0 0]
      link override fft_stage_8/sync_delay_x/Relational: xl_area=[1 0 0 2 0 0 0]
      link override fft_stage_8/sync_delay_x/Relational1: xl_area=[1 0 0 2 0 0 0]
      link override fft_stage_9/Counter: xl_area=[1 2 0 2 0 0 0]
      link override fft_stage_9/Delay: xl_area=[1 1 0 0 0 0 0]
      link override fft_stage_9/Logical1: xl_area=[1 1 0 1 0 0 0]
      link override fft_stage_9/Mux: xl_area=[18 36 0 36 0 0 0]
      link override fft_stage_9/Mux1: xl_area=[18 36 0 36 0 0 0]
      link override fft_stage_9/butterfly/AddSub: xl_area=[12 23 0 23 0 0 0]
      link override fft_stage_9/butterfly/AddSub1: xl_area=[12 23 0 23 0 0 0]
      link override fft_stage_9/butterfly/AddSub2: xl_area=[12 23 0 23 0 0 0]
      link override fft_stage_9/butterfly/AddSub3: xl_area=[12 23 0 23 0 0 0]
      link override fft_stage_9/butterfly/Convert: xl_area=[31 18 0 61 0 0 0]
      link override fft_stage_9/butterfly/Convert1: xl_area=[31 18 0 61 0 0 0]
      link override fft_stage_9/butterfly/Convert2: xl_area=[31 18 0 61 0 0 0]
      link override fft_stage_9/butterfly/Convert3: xl_area=[31 18 0 61 0 0 0]
      link override fft_stage_9/butterfly/Delay: xl_area=[1 1 0 1 0 0 0]
      link override fft_stage_9/butterfly/Delay3: xl_area=[1 1 0 0 0 0 0]
      link override fft_stage_9/butterfly/Inverter: xl_area=[0 0 0 0 0 0 0]
      link override fft_stage_9/butterfly/Logical: xl_area=[1 1 0 1 0 0 0]
      link override fft_stage_9/butterfly/Logical1: xl_area=[1 1 0 1 0 0 0]
      link override fft_stage_9/butterfly/Logical10: xl_area=[1 1 0 1 0 0 0]
      link override fft_stage_9/butterfly/Logical11: xl_area=[1 1 0 1 0 0 0]
      link override fft_stage_9/butterfly/Logical12: xl_area=[1 1 0 1 0 0 0]
      link override fft_stage_9/butterfly/Logical13: xl_area=[1 1 0 1 0 0 0]
      link override fft_stage_9/butterfly/Logical2: xl_area=[1 1 0 1 0 0 0]
      link override fft_stage_9/butterfly/Logical3: xl_area=[1 1 0 1 0 0 0]
      link override fft_stage_9/butterfly/Logical4: xl_area=[1 1 0 1 0 0 0]
      link override fft_stage_9/butterfly/Logical5: xl_area=[1 1 0 1 0 0 0]
      link override fft_stage_9/butterfly/Logical6: xl_area=[1 1 0 1 0 0 0]
      link override fft_stage_9/butterfly/Logical7: xl_area=[1 1 0 1 0 0 0]
      link override fft_stage_9/butterfly/Logical8: xl_area=[1 1 0 1 0 0 0]
      link override fft_stage_9/butterfly/Logical9: xl_area=[1 1 0 1 0 0 0]
      link override fft_stage_9/butterfly/Mux: xl_area=[12 24 0 24 0 0 0]
      link override fft_stage_9/butterfly/Mux1: xl_area=[12 24 0 24 0 0 0]
      link override fft_stage_9/butterfly/Mux2: xl_area=[12 24 0 24 0 0 0]
      link override fft_stage_9/butterfly/Mux3: xl_area=[12 24 0 24 0 0 0]
      link override fft_stage_9/butterfly/twiddle_general/AddSub: xl_area=[11 21 0 21 0 0 0]
      link override fft_stage_9/butterfly/twiddle_general/AddSub1: xl_area=[11 21 0 21 0 0 0]
      link override fft_stage_9/butterfly/twiddle_general/Convert: xl_area=[0 0 0 0 0 0 0]
      link override fft_stage_9/butterfly/twiddle_general/Convert1: xl_area=[0 0 0 0 0 0 0]
      link override fft_stage_9/butterfly/twiddle_general/Convert2: xl_area=[0 0 0 0 0 0 0]
      link override fft_stage_9/butterfly/twiddle_general/Convert3: xl_area=[0 0 0 0 0 0 0]
      link override fft_stage_9/butterfly/twiddle_general/Delay: xl_area=[18 36 0 36 0 0 0]
      link override fft_stage_9/butterfly/twiddle_general/Delay1: xl_area=[18 36 0 0 0 0 0]
      link override fft_stage_9/butterfly/twiddle_general/Delay2: xl_area=[1 1 0 1 0 0 0]
      link override fft_stage_9/butterfly/twiddle_general/Mult: xl_area=[36 72 0 36 0 1 0]
      link override fft_stage_9/butterfly/twiddle_general/Mult1: xl_area=[36 72 0 36 0 1 0]
      link override fft_stage_9/butterfly/twiddle_general/Mult2: xl_area=[36 72 0 36 0 1 0]
      link override fft_stage_9/butterfly/twiddle_general/Mult3: xl_area=[36 72 0 36 0 1 0]
      link override fft_stage_9/butterfly/twiddle_general/br_coeff_gen/Counter: xl_area=[5 9 0 9 0 0 0]
      link override fft_stage_9/butterfly/twiddle_general/br_coeff_gen/ROM: xl_area=[0 0 1 0 0 0 0]
      link override fft_stage_9/butterfly/twiddle_general/br_coeff_gen/ROM1: xl_area=[0 0 1 0 0 0 0]
      link override fft_stage_9/butterfly/twiddle_general_3mult/AddSub: xl_area=[11 22 0 22 0 0 0]
      link override fft_stage_9/butterfly/twiddle_general_3mult/AddSub1: xl_area=[10 19 0 19 0 0 0]
      link override fft_stage_9/butterfly/twiddle_general_3mult/AddSub2: xl_area=[10 19 0 19 0 0 0]
      link override fft_stage_9/butterfly/twiddle_general_3mult/AddSub3: xl_area=[10 19 0 19 0 0 0]
      link override fft_stage_9/butterfly/twiddle_general_3mult/AddSub4: xl_area=[11 22 0 22 0 0 0]
      link override fft_stage_9/butterfly/twiddle_general_3mult/Convert: xl_area=[0 0 0 0 0 0 0]
      link override fft_stage_9/butterfly/twiddle_general_3mult/Convert1: xl_area=[0 0 0 0 0 0 0]
      link override fft_stage_9/butterfly/twiddle_general_3mult/Convert2: xl_area=[0 0 0 0 0 0 0]
      link override fft_stage_9/butterfly/twiddle_general_3mult/Convert3: xl_area=[0 0 0 0 0 0 0]
      link override fft_stage_9/butterfly/twiddle_general_3mult/Convert4: xl_area=[0 0 0 0 0 0 0]
      link override fft_stage_9/butterfly/twiddle_general_3mult/Convert5: xl_area=[0 0 0 0 0 0 0]
      link override fft_stage_9/butterfly/twiddle_general_3mult/Delay: xl_area=[18 36 0 36 0 0 0]
      link override fft_stage_9/butterfly/twiddle_general_3mult/Delay1: xl_area=[18 36 0 0 0 0 0]
      link override fft_stage_9/butterfly/twiddle_general_3mult/Delay2: xl_area=[1 1 0 1 0 0 0]
      link override fft_stage_9/butterfly/twiddle_general_3mult/Delay3: xl_area=[9 18 0 0 0 0 0]
      link override fft_stage_9/butterfly/twiddle_general_3mult/Delay4: xl_area=[9 18 0 0 0 0 0]
      link override fft_stage_9/butterfly/twiddle_general_3mult/Delay5: xl_area=[9 18 0 0 0 0 0]
      link override fft_stage_9/butterfly/twiddle_general_3mult/Mult: xl_area=[36 72 0 36 0 1 0]
      link override fft_stage_9/butterfly/twiddle_general_3mult/Mult1: xl_area=[36 72 0 36 0 1 0]
      link override fft_stage_9/butterfly/twiddle_general_3mult/Mult2: xl_area=[36 72 0 36 0 1 0]
      link override fft_stage_9/butterfly/twiddle_general_3mult/br_coeff_gen/Counter: xl_area=[5 9 0 9 0 0 0]
      link override fft_stage_9/butterfly/twiddle_general_3mult/br_coeff_gen/ROM: xl_area=[0 0 1 0 0 0 0]
      link override fft_stage_9/butterfly/twiddle_general_3mult/br_coeff_gen/ROM1: xl_area=[0 0 1 0 0 0 0]
      link override fft_stage_9/delay_b/delay_im/delay_slr/delay_slr: xl_area=[9 18 0 18 0 0 0]
      link override fft_stage_9/delay_b/delay_re/delay_slr/delay_slr: xl_area=[9 18 0 18 0 0 0]
      link override fft_stage_9/delay_b/delay_slr/delay_slr: xl_area=[18 36 0 36 0 0 0]
      link override fft_stage_9/delay_f/delay_im/delay_slr/delay_slr: xl_area=[9 18 0 18 0 0 0]
      link override fft_stage_9/delay_f/delay_re/delay_slr/delay_slr: xl_area=[9 18 0 18 0 0 0]
      link override fft_stage_9/delay_f/delay_slr/delay_slr: xl_area=[18 36 0 36 0 0 0]
      link override fft_stage_9/sync_delay_x/Counter: xl_area=[2 2 0 3 0 0 0]
      link override fft_stage_9/sync_delay_x/Logical: xl_area=[1 0 0 1 0 0 0]
      link override fft_stage_9/sync_delay_x/Mux: xl_area=[1 0 0 1 0 0 0]
      link override fft_stage_9/sync_delay_x/Relational: xl_area=[1 0 0 1 0 0 0]
      link override fft_stage_9/sync_delay_x/Relational1: xl_area=[1 0 0 1 0 0 0]
  wires:
  Gateway In1/1 -> biplex_core/1
  Gateway In2/1 -> biplex_core/2
  Gateway In3/1 -> biplex_core/3
  Constant4/1 -> biplex_core/4
  biplex_core/1 -> Gateway Out/1
  biplex_core/2 -> Gateway Out1/1
  biplex_core/3 -> Gateway Out2/1
  biplex_core/4 -> Gateway Out3/1
  Constant6/1 -> Gateway In1/1
  Constant8/1 -> Gateway In2/1
  Constant10/1 -> Gateway In3/1
  Gateway Out/1 -> Terminator/1
  Gateway Out1/1 -> Terminator2/1
  Gateway Out2/1 -> Terminator4/1
  Gateway Out3/1 -> Terminator6/1
